simulink model "AUAV_V3_TestSensors_"  (R2015a)
settings: Solver=FixedStepDiscrete  StartTime=0.0  StopTime=10.0  FixedStep=T  RelTol=1e-3
PreLoadFcn:
  | %T = 0.0025;
  | MavlinkBus;
  | mcuInit;
  | % Baro Altitude Computation
  | % =========================
  | basePressure = 98192.64;
  | baseTemp = 288.215;
  | lapseRate = -0.00198122;
  | baseHeight = 0;
values from neighbouring files (symbols this model uses):
  apSampleTime = 0.01    [mcuInit.m]
  latlong_WP = 1    [mcuInit.m]
  mavlink_attitude_t = Simulink.Bus    [MavlinkBusMarcello.m]
  mavlink_gps_raw_int_t = Simulink.Bus    [MavlinkBus.m]    (also in MavlinkBusMarcello.m)
  mavlink_raw_imu_t = Simulink.Bus    [MavlinkBus.m]    (also in MavlinkBusMarcello.m)
  mavlink_scaled_pressure_t = Simulink.Bus    [MavlinkBus.m]    (also in MavlinkBusMarcello.m)
  mavlink_servo_output_raw_t = Simulink.Bus    [MavlinkBusMarcello.m]
  mavlink_sys_status_t = Simulink.Bus    [MavlinkBus.m]    (also in MavlinkBusMarcello.m)
  T = 0.01    [mcuInit.m]
  Xpoints = [0 0]    [mcuInit.m]
  Ypoints = [0 0]    [mcuInit.m]
  Zpoints = [0 0]    [mcuInit.m]
undefined symbols (not defined in the file or in its folder): A0, A14, A15, A2, A3, A4, A5, A6, accBiasRateLimit, B0, bankCommandLimit, barAdjust, baroCutoff, baroCutTemp, cubeAccelGain16405, cubeGyroGain16405, cubeMagGain16405, D0, D11, D7, D8, daLimit, data, daTrimMax, daTrimMin, deLimit, deTrimMax, deTrimMin, drLimit, drTrimMax, drTrimMin, dtLimit, dtTrimMax, dtTrimMin, F2, F3, G0, G13, G15, gaind, GS_location, gyroBiasRateLimit, IC1max, IPStar, ISA_g, Max, maxAcc, MaxDwnPthStar, maxDynPressure, maxEta, mlParamInterface, ms, OC1max, P112, P125, P127, P16, P20, P21, P30 ... (+26)
undefined symbols (not defined in the file): baroOffset, baroScale, barTGain1, barTGain2, barTMean1, barTMean2, bda, bde, bdr, bdt, bICda, bICde, bICdr, bICdt, derivativesConstant, lowRateSensorCutoff, mainSensorCutoff, mda, mde, mdr, mdt, mICda, mICde, mICdr, mICdt, pitotOffset, pitotScale, pitTGain1, pitTGain2, pitTMean1, pitTMean2, powerOffset, powerScale, pressureSensorCutoff, tempOffset, tempScale, vzCutoff, xCutoff, yCutoff
libraries: MCHP_Blockset x150, simulink x84, SLUGS_Library x31, aerolibconvert2 x6, aerolibutil x4, aerolibtransform2 x3, dspmtrx3 x2, aerolibobsolete x2
(part 1 of 20)
Description:
  | Rapid Prototyping model.
  | Require the MPLAB Blockset for Simulink v3.30 or above. [http://www.microchip.com/SimulinkBlocks]
  | Author:Avi Manor Based on Lubin Kerhuels work and code from SLUGS
  | 
  | Test Mavlink on AUAV V3 board from Asrovtech. [http://arsovtech.com/?p=1414]
settings Model: Creator=M91449  LastModifiedBy=User
settings DataIOCC: SignalLoggingSaveFormat=ModelDataLogs
settings OptimizationCC: InlineParams=on  InlineInvariantSignals=on  EnhancedBackFolding=on  OptimizeModelRefInitCode=on  LifeSpan=1
settings DebuggingCC: UnderspecifiedInitializationDetection=Classic  MergeDetectMultiDrivingBlocksExec=none  SolverPrmCheckMsg=warning  MultiTaskDSMMsg=none  FcnCallInpInsideContextMsg=EnableAllAsWarning
settings HardwareCC: ProdBitPerInt=16  ProdBitPerPointer=16  ProdLargestAtomicInteger=Integer  ProdIntDivRoundTo=Zero  ProdEndianess=LittleEndian  ProdWordSize=16  ProdHWDeviceType=Generic->Custom
settings RTWCC: SystemTargetFile=MCHP_dsPIC_stf.tlc  GenCodeOnly=on  TemplateMakefile=MCHP_dsPIC.tmf  Description=Microchip Embedded Target PIC24 dsPIC30 dsPIC33 (real-time)  CustomHeaderCode="#include \"MavlinkComm.h\""
settings RTWCC: CustomSourceCode=|
  | #include "gpsPort.h"
  | #include "MavlinkComm.h"
settings RTWCC: CustomInclude=|
  | mavlink/include/slugs
  | clib\
settings RTWCC: CustomSource=|
  | clib/circBuffer.c
  | clib/gpsPort.c
  | clib/gpsUblox.c
  | clib/MavlinkComm.c
  | clib/apUtils.c
  | clib/mavlinkCommsControlMcu.c
  | clib/mavlinkControlMcu.c
  | clib/mavlinkSensorMcu.c
  | clib/updateControlMcuState.c
  | clib/updateSensorMcuState.c
  | clib/novatel.c
  | clib/navSupport.c
  | clib/hil.c
  | clib/adisCube16405.c
settings RTWCC: CustomInitializer=|
  | uartBufferInit();
  | uartMavlinkBufferInit ();
  | InitParameterInterface();
settings CodeAppCC: IgnoreCustomStorageClasses=off  InternalIdentifier=Classic
settings STFCustomTargetCC: TargetLibSuffix=_lib.a  GenerateSampleERTMain=off  IncludeMdlTerminateFcn=off  CombineOutputUpdateFcns=on  SuppressErrorStatus=on  SupportContinuousTime=off  SupportNonInlinedSFcns=on  SupportVariableSizeSignals=off  SystemTargetFile=MCHP_dsPIC_stf.tlc
settings ERTTargetCC: TargetLibSuffix=_lib.a  GenerateSampleERTMain=off  IncludeMdlTerminateFcn=off  SuppressErrorStatus=on  SupportContinuousTime=off  SupportNonInlinedSFcns=on  SupportVariableSizeSignals=off  ExtModeMexFile=ext_serial_win32_comm_no_acks_rtt  ExtModeMexArgs=1 4 57600  ERTSrcFileBannerTemplate=MCHP_dsPIC_code_template.cgt  ERTHdrFileBannerTemplate=MCHP_dsPIC_code_template.cgt  ERTDataSrcFileTemplate=MCHP_dsPIC_code_template.cgt  ERTDataHdrFileTemplate=MCHP_dsPIC_code_template.cgt  ERTCustomFileTemplate=MCHP_main.tlc

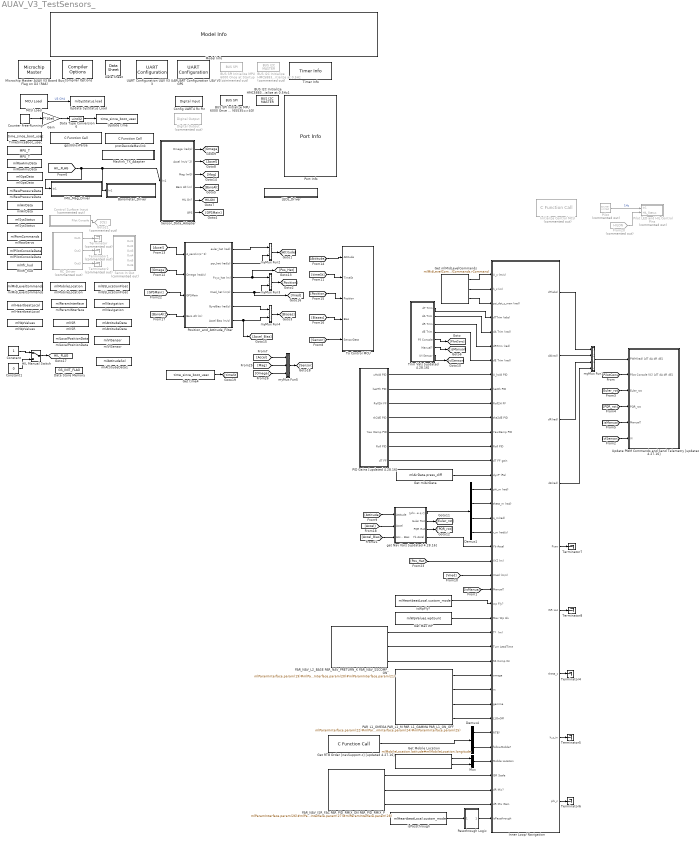
== system AUAV_V3_TestSensors_ ==
  " gpsUbloxParse" : MCHP_Blockset/User Functions/C Function Call  ParseFilesChkbx=on  ListFunctions1=Custom Function  Function1=void gpsUbloxParse(void)  AddHeaderDeclaration=on  Function1Type=when block is updated (default)  FctReturnBlockOut=on  DataCollected="s.chksm=reshape({ '638503-Feb-2015 20:58:10','251913-Sep-2016 12:15:14','1628414-Sep-2016 10:06:29','3596013-Sep-2016 14:21:45','360317-Jun-2016 15:34:16','7112612-Sep-2016 14:50:45','954931-Aug-2016 15:03:40','295329-Aug-2016 11:32:53','268124-Jun-2016 00:23:34','556017-Jun-2016 15:34:16','963217-Jun-2016 15:34:16','1086024-Jun-2016 00:23:34','358817-Jun-2016 15:34:16','985917-Jun-2016 15:34:16','481613-Sep-2016 14:21:38'},1,15);s.File1=reshape({ '  void  newCircBuffer(CBRef cB)','  void  freeCircBuffer(CBRef* cB)','  void  freeCircBuffer(CBRef* cB)',' unsigned int  getLength(CBRef cB)','  int  readHead(CBRef cB)','  int  readTail(CBRef cB)',' unsigned char  peak(CBRef cB)',' unsigned char  readFront(CBRef cB)',' unsigned char  writeBack(CBRef cB, unsigned char data)','  void  makeEmpty(CBRef cB)','  void  printCircBuf(CBRef cB)'},1,11);s.File2=reshape({ '  void  uartBufferInit(void)','  void  __attribute__((__interrupt__, no_auto_psv)) _U4RXInterrupt(void)','  void  getGPSRawData(unsigned char* gpsBuffer)',' unsigned char  isGPSNovatel(void)'},1,4);s.File3=reshape({ '  char  hex2char(char halfhex)','  float  degMinToDeg(unsigned char degrees, float minutes)',' unsigned char  gpsUbloxSeparate(unsigned char* outStream)','  void  gpsUbloxParse(void)','  void  getGpsUbloxMainData(float* data)','  char  gpSmbl(char symbl)',' unsigned char  myTokenizer(char* stringToTokenize, char token, char * returnToken)','  void  parseRMC(unsigned char* stream)','  void  parseGGA(unsigned char* stream)',' unsigned char  getChecksum(unsigned char* sentence, unsigned char size)','  void  gpsDebugMsg(unsigned char buf)'},1,11);s.File4=reshape({ '  void  uartMavlinkBufferInit(void)','  void __attribute__((__interrupt__,__auto_psv__)) _U1RXInterrupt(void)','  uint8_t  isFinite(float s)','  void  InitParameterInterface(void)','  void  protDecodeMavlink(void)','  uint16_t  MissionInterfaceResponse(uint8_t system_id, uint8_t component_id)','  uint16_t  ParameterInterfaceResponse(uint8_t system_id, uint8_t component_id)','  uint16_t  PackHeartBeat(uint8_t system_id, uint8_t component_id)','  uint16_t  PackTextMsg(uint8_t system_id, uint8_t component_id, unsigned char buf)','  uint16_t  PackRawIMU(uint8_t system_id, uint8_t component_id, mavlink_raw_imu_t mlRawIMUData ,uint32_t time_usec)','  uint16_t  PackGpsRawInt(uint8_t system_id, uint8_t component_id, mavlink_gps_raw_int_t mlRawGpsDataInt)','  uint16_t  PackScaledPressure(uint8_t system_id, uint8_t component_id, mavlink_scaled_pressure_t mlAirData ,uint32_t time_usec)','  uint16_t  PackSysStatus(uint8_t system_id, uint8_t component_id, mavlink_sys_status_t mlSysStatus)','  uint16_t  PackRawServo(uint8_t system_id, uint8_t component_id, mavlink_servo_output_raw_t mlPwmCommands ,uint32_t time_usec)','  uint16_t  PackRawRC(uint8_t system_id, uint8_t component_id, mavlink_rc_channels_raw_t mlRC_Commands ,uint32_t time_usec)','  uint16_t  PackVFR_HUD(uint8_t system_id, uint8_t component_id, mavlink_vfr_hud_t mlVfr_hud ,uint32_t time_usec)','  char  sendQGCDebugMessage(const char * dbgMessage, char severity, unsigned char* bytesToAdd, char positionStart)','  void  TxN_Data_OverU1(uint16_t N)'},1,18);s.File5=reshape({ '  float  myAtan2(float num, float denom)','  float  myPow(float x, float toTheN)','  float  mySqrt(float x)','  float  myAbs(float x)','  float  myAtan(float x)','  float  myAsin(float x)','  float  mySin(float x)','  float  myCos(float x)','  float  myTan(float x)','  float  myAcos(float x)','  float  myExp(float x)','  void  hugeDelay(void)','  void  smallDelay(void)','  void  tinyDelay(void)','  void  printToUart2(const char *fmt, ...)'},1,15);s.File6=reshape({ '  void  sendTelemetryMavlink(unsigned char* dataOut)','  void  uart2Init(void)','  void  gsRead(unsigned char* gsChunk)','  void  prepareTelemetryMavlink(unsigned char* dataOut)','  void  prepareTelemetryMavlink(unsigned char* dataOut)','  void  sendTelemetryMavlink(unsigned char* dataOut)','  void  copyBufferToDMA1(unsigned char size)','  void  send2GS(unsigned char* protData)','  uint8_t  clearWaypointsFrom(uint8_t startingWp)','  void  addMessageToSpiOut(mavlink_message_t* msg)'},1,10);s.File7={ '  void  populateParameterInterface(void)'};s.File8={ '  void  mavlinkInit(void)'};s.File9=reshape({ '  void  updatePWM(unsigned short * PWMData)','  void  updatePWMTrim(unsigned short PWMData, unsigned char channel)','  void  updateLoad(uint8_t mcuLoad)','  void  updateEuler(float* newEuler)','  void  updatePQR(float* newPQR)',' unsigned char  getHilOnOff(void)','  uint8_t  getLightsOnOff(void)','  uint8_t  getLightsDayNight(void)','  void  updateVISensor(uint16_t* data)','  void  updatePTZ(int16_t* ptz)'},1,10);s.File10=reshape({ '  void  updateRawADCData(int16_t* adcData)','  void  updateAirData(float* airData)','  void  updateLoadData(uint8_t load, uint16_t mvPower)','  void  updateAttitude(float * attitudeData)','  void  getGSLocation(float* altLatLon)','  void  updateTimeStamp(uint32_t timeSt)','  void  updatePosition(float * posData)','  void  updatePilotConsole(uint16_t * pilData)','  void  updateDiagnosticFl(float* diagFl)','  void  updateDiagnosticSh(int16_t* diagSh)','  void  updateBias(float * biasData)','  void  updateSensorData(float* sens)','  uint8_t  isFixValid(void)','  void  updateSensorDiag(float* diag)'},1,14);s.File11=reshape({ '  void  gpsInit(void)','  void  gpsParse(uint8_t* dataStream)','  void  updateStatus(uint8_t* completeMessage)','  void  updatePositionData(uint8_t* completeMessage)','  void  updateVelocityData(uint8_t* completeMessage)','  void  updateTimeData(uint8_t* completeMessage)','  void  getGpsMainData(float* data)','  uint32_t  CRC32Value(int32_t i)','  uint32_t  CalculateBlockCRC32(uint32_t ulCount, uint8_t *ucBuffer)','  uint16_t  charsToUint16(uint8_t* data)','  uint32_t  charsToUint32(uint8_t* data)','  float  charsToFloat(uint8_t* data)','  double  charsToDouble(uint8_t* data)'},1,13);s.File12=reshape({ '  void  getMidLevelCommands(float* commands)',' unsigned char  isApManual(uint16_t failsafe)','  float  getParamIdx(unsigned char idx)','  void  getRangeOfParams(uint8_t startIdx, uint8_t endIdx, float* parameters)','  float  getDynamic(void)','  void  getAttitude(float* attitude)','  void  getXYZ(float* xyz)','  void  getVned(float* xyz)','  uint8_t  getMaxWp(void)',' unsigned char  isWpFly(void)',' unsigned char  isPassthrough(void)','  void  setDiagnosticFloat(float * flValues)','  void  setDiagnosticShort(int16_t* shValues)','  void  getWP(unsigned char idx, float* WPpos)','  void  setLogFloat1(float * flValues)','  void  setLogFloat2(float * flValues)',' unsigned char  getApControlType(void)',' unsigned char  getPassValues(uint8_t* pasVals)','  void  setCurrentCommands(float airSpeed)','  void  getCurrentGPSPos(float* latLonAlt)','  void  setNavLong(float* values)','  void  setNavLat(float* values)','  void  setNavNav(float* values)','  void  getAccels(float * accels)','  void  getAccBias(float * bias)','  void  getRTB(uint8_t* rtb)','  void  getMobileLocation(float* loc)','  uint8_t  getNavMode(void)','  void  getISRLocation(float* loc)','  uint8_t  getISRCameraOption1(void)',' unsigned short  meanFilter5(unsigned short * values)','  uint8_t  justEnabled(uint8_t enableValue, uint8_t index)',' unsigned char  quickSort(unsigned short *arr, char elements)'},1,33);s.File13=reshape({ '  void  hilRead(unsigned char* hilChunk)','  void  hil_getRawRead(short * rawData)','  void  hil_getVned(float* vned)','  void  hil_getEuler(float* euler)','  void  hil_getRates(float* pqr)','  void  hil_getXYZ(float* xyz)',' unsigned int  hil_getTs(void)','  void  protDecodeHil(uint8_t* dataIn)'},1,8);s.File14=reshape({ '  void  cubeInit(void)','  void  getCubeData(short * cubeData)','  void  updateCubeData(void)','  int16_t  averageData(int16_t* theData, uint8_t count)',' unsigned short  write2Cube(unsigned short data2Send)','  void  __attribute__((interrupt, no_auto_psv)) _T5Interrupt(void)','  short  convert14BitToShort(short wordData)','  short  convert12BitToShort(short wordData)',' unsigned char  isCube16405(void)'},1,9);s.File15=reshape({ '  void  uartMavlinkBufferInit(void)','  uint16_t  PackHeartBeat(uint8_t system_id, uint8_t component_id)','  uint16_t  PackRawRC(uint8_t system_id, uint8_t component_id, mavlink_rc_channels_raw_t mlRC_Commands, uint32_t time_usec)','  uint16_t  PackVFR_HUD(uint8_t system_id, uint8_t component_id, mavlink_vfr_hud_t mlVfr_hud, uint32_t time_usec)','  uint16_t  PackRawIMU(uint8_t system_id, uint8_t component_id, mavlink_raw_imu_t mlRawIMUData ,uint32_t time_usec)','  char  sendQGCDebugMessage(const char * dbgMessage, char severity, unsigned char* bytesToAdd, char positionStart)','  uint16_t  PackGpsRawInt(uint8_t system_id, uint8_t component_id, mavlink_gps_raw_int_t mlRawGpsDataInt)','  uint16_t  PackScaledPressure(uint8_t system_id, uint8_t component_id, mavlink_scaled_pressure_t mlAirData, uint32_t time_usec)','  uint16_t  PackSysStatus(uint8_t system_id, uint8_t component_id, mavlink_sys_status_t mlSysStatus)'},1,9);"  ORDERING=None  SampleTime=0.5  MCHP_MASTERLINK=|  PinDigitalInput=[]  PinDigitalOutput=[]  PinAnalogInput=[]
      | AUAV_V3_TestSensors_/Microchip Master
      | AUAV V3 Board
      | Busy Flag on D2 (RA6)
  " protDecodeMavlink" : MCHP_Blockset/User Functions/C Function Call  ParseFilesChkbx=on  ListFunctions1=Custom Function  Function1=void protDecodeMavlink(void)  AddHeaderDeclaration=off  Function1Type=when block is updated (default)  FctReturnBlockOut=on  DataCollected="s.chksm=reshape({ '638503-Feb-2015 20:58:10','251913-Sep-2016 12:15:14','1628414-Sep-2016 10:06:29','3754120-Sep-2016 14:41:10','360317-Jun-2016 15:34:16','7114620-Sep-2016 10:38:54','954931-Aug-2016 15:03:40','296127-Sep-2016 09:37:43','268124-Jun-2016 00:23:34','556017-Jun-2016 15:34:16','963217-Jun-2016 15:34:16','1086024-Jun-2016 00:23:34','372414-Sep-2016 14:01:55','998814-Sep-2016 11:55:45','509015-Sep-2016 09:12:19'},1,15);s.File1=reshape({ '  void  newCircBuffer(CBRef cB)','  void  freeCircBuffer(CBRef* cB)','  void  freeCircBuffer(CBRef* cB)',' unsigned int  getLength(CBRef cB)','  int  readHead(CBRef cB)','  int  readTail(CBRef cB)',' unsigned char  peak(CBRef cB)',' unsigned char  readFront(CBRef cB)',' unsigned char  writeBack(CBRef cB, unsigned char data)','  void  makeEmpty(CBRef cB)','  void  printCircBuf(CBRef cB)'},1,11);s.File2=reshape({ '  void  uartBufferInit(void)','  void  __attribute__((__interrupt__, no_auto_psv)) _U4RXInterrupt(void)','  void  getGPSRawData(unsigned char* gpsBuffer)',' unsigned char  isGPSNovatel(void)'},1,4);s.File3=reshape({ '  char  hex2char(char halfhex)','  float  degMinToDeg(unsigned char degrees, float minutes)',' unsigned char  gpsUbloxSeparate(unsigned char* outStream)','  void  gpsUbloxParse(void)','  void  getGpsUbloxMainData(float* data)','  char  gpSmbl(char symbl)',' unsigned char  myTokenizer(char* stringToTokenize, char token, char * returnToken)','  void  parseRMC(unsigned char* stream)','  void  parseGGA(unsigned char* stream)',' unsigned char  getChecksum(unsigned char* sentence, unsigned char size)','  void  gpsDebugMsg(unsigned char buf)'},1,11);s.File4=reshape({ '  void  uartMavlinkBufferInit(void)','  void __attribute__((__interrupt__,__auto_psv__)) _U1RXInterrupt(void)','  uint8_t  isFinite(float s)','  void  InitParameterInterface(void)','  void  protDecodeMavlink(void)','  uint16_t  MissionInterfaceResponse(uint8_t system_id, uint8_t component_id)','  uint16_t  ParameterInterfaceResponse(uint8_t system_id, uint8_t component_id)','  uint16_t  PackHeartBeat(uint8_t system_id, uint8_t component_id)','  uint16_t  PackTextMsg(uint8_t system_id, uint8_t component_id, unsigned char buf)','  uint16_t  PackRawIMU(uint8_t system_id, uint8_t component_id, mavlink_raw_imu_t mlRawIMUData ,uint32_t time_usec)','  uint16_t  PackGpsRawInt(uint8_t system_id, uint8_t component_id, mavlink_gps_raw_int_t mlRawGpsDataInt ,uint32_t time_usec)','  uint16_t  PackScaledPressure(uint8_t system_id, uint8_t component_id, mavlink_scaled_pressure_t mlAirData ,uint32_t time_usec)','  uint16_t  PackSysStatus(uint8_t system_id, uint8_t component_id, mavlink_sys_status_t mlSysStatus)','  uint16_t  PackRawServo(uint8_t system_id, uint8_t component_id, mavlink_servo_output_raw_t mlPwmCommands ,uint32_t time_usec)','  uint16_t  HIL_PackRawServo(uint8_t system_id, uint8_t component_id, mavlink_servo_output_raw_t mlPwmCommands ,uint32_t time_usec)','  uint16_t  PackRawRC(uint8_t system_id, uint8_t component_id, mavlink_rc_channels_raw_t mlRC_Commands ,uint32_t time_usec)','  uint16_t  PackVFR_HUD(uint8_t system_id, uint8_t component_id, mavlink_vfr_hud_t mlVfr_hud ,uint32_t time_usec)','  char  sendQGCDebugMessage(const char * dbgMessage, char severity, unsigned char* bytesToAdd, char positionStart)','  void  TxN_Data_OverU1(uint16_t N)','  void  TxN_Data_OverU4(uint16_t N)'},1,20);s.File5=reshape({ '  float  myAtan2(float num, float denom)','  float  myPow(float x, float toTheN)','  float  mySqrt(float x)','  float  myAbs(float x)','  float  myAtan(float x)','  float  myAsin(float x)','  float  mySin(float x)','  float  myCos(float x)','  float  myTan(float x)','  float  myAcos(float x)','  float  myExp(float x)','  void  hugeDelay(void)','  void  smallDelay(void)','  void  tinyDelay(void)','  void  printToUart2(const char *fmt, ...)'},1,15);s.File6=reshape({ '  void  sendTelemetryMavlink(unsigned char* dataOut)','  void  uart2Init(void)','  void  gsRead(unsigned char* gsChunk)','  void  prepareTelemetryMavlink(unsigned char* dataOut)','  void  prepareTelemetryMavlink(unsigned char* dataOut)','  void  sendTelemetryMavlink(unsigned char* dataOut)','  void  copyBufferToDMA1(unsigned char size)','  void  send2GS(unsigned char* protData)','  uint8_t  clearWaypointsFrom(uint8_t startingWp)','  void  addMessageToSpiOut(mavlink_message_t* msg)'},1,10);s.File7={ '  void  populateParameterInterface(void)'};s.File8={ '  void  mavlinkInit(void)'};s.File9=reshape({ '  void  updatePWM(unsigned short * PWMData)','  void  updatePWMTrim(unsigned short PWMData, unsigned char channel)','  void  updateLoad(uint8_t mcuLoad)','  void  updateEuler(float* newEuler)','  void  updatePQR(float* newPQR)',' unsigned char  getHilOnOff(void)','  uint8_t  getLightsOnOff(void)','  uint8_t  getLightsDayNight(void)','  void  updateVISensor(uint16_t* data)','  void  updatePTZ(int16_t* ptz)'},1,10);s.File10=reshape({ '  void  updateRawADCData(int16_t* adcData)','  void  updateAirData(float* airData)','  void  updateLoadData(uint8_t load, uint16_t mvPower)','  void  updateAttitude(float * attitudeData)','  void  getGSLocation(float* altLatLon)','  void  updateTimeStamp(uint32_t timeSt)','  void  updatePosition(float * posData)','  void  updatePilotConsole(uint16_t * pilData)','  void  updateDiagnosticFl(float* diagFl)','  void  updateDiagnosticSh(int16_t* diagSh)','  void  updateBias(float * biasData)','  void  updateSensorData(float* sens)','  uint8_t  isFixValid(void)','  void  updateSensorDiag(float* diag)'},1,14);s.File11=reshape({ '  void  gpsInit(void)','  void  gpsParse(uint8_t* dataStream)','  void  updateStatus(uint8_t* completeMessage)','  void  updatePositionData(uint8_t* completeMessage)','  void  updateVelocityData(uint8_t* completeMessage)','  void  updateTimeData(uint8_t* completeMessage)','  void  getGpsMainData(float* data)','  uint32_t  CRC32Value(int32_t i)','  uint32_t  CalculateBlockCRC32(uint32_t ulCount, uint8_t *ucBuffer)','  uint16_t  charsToUint16(uint8_t* data)','  uint32_t  charsToUint32(uint8_t* data)','  float  charsToFloat(uint8_t* data)','  double  charsToDouble(uint8_t* data)'},1,13);s.File12=reshape({ '  void  getMidLevelCommands(float* commands)',' unsigned char  isApManual(uint16_t failsafe)','  float  getParamIdx(unsigned char idx)','  void  getRangeOfParams(uint8_t startIdx, uint8_t endIdx, float* parameters)','  float  getDynamic(void)','  void  getAttitude(float* attitude)','  void  getXYZ(float* xyz)','  void  getVned(float* xyz)','  uint8_t  getMaxWp(void)',' unsigned char  isWpFly(void)',' unsigned char  isPassthrough(void)','  void  setDiagnosticFloat(float * flValues)','  void  setDiagnosticShort(int16_t* shValues)','  void  getWP(unsigned char idx, float* WPpos)','  void  setLogFloat1(float * flValues)','  void  setLogFloat2(float * flValues)',' unsigned char  getApControlType(void)',' unsigned char  getPassValues(uint8_t* pasVals)','  void  setCurrentCommands(float airSpeed)','  void  getCurrentGPSPos(float* latLonAlt)','  void  setNavLong(float* values)','  void  setNavLat(float* values)','  void  setNavNav(float* values)','  void  getAccels(float * accels)','  void  getAccBias(float * bias)','  void  getRTB(uint8_t* rtb)','  void  getMobileLocation(float* loc)','  uint8_t  getNavMode(void)','  void  getISRLocation(float* loc)','  uint8_t  getISRCameraOption1(void)',' unsigned short  meanFilter5(unsigned short * values)','  uint8_t  justEnabled(uint8_t enableValue, uint8_t index)',' unsigned char  quickSort(unsigned short *arr, char elements)'},1,33);s.File13=reshape({ '  void  hilRead(unsigned char* hilChunk)','  void  hil_getRawRead(short * rawData)','  void  hil_getVned(float* vned)','  void  hil_getEuler(float* euler)','  void  hil_getRates(float* pqr)','  void  hil_getXYZ(float* xyz)',' unsigned int  hil_getTs(void)','  void  protDecodeHil(uint8_t* dataIn)'},1,8);s.File14=reshape({ '  void  cubeInit(void)','  void  getCubeData(short * cubeData)','  void  updateCubeData(void)','  int16_t  averageData(int16_t* theData, uint8_t count)',' unsigned short  write2Cube(unsigned short data2Send)','  short  convert14BitToShort(short wordData)','  short  convert12BitToShort(short wordData)',' unsigned char  isCube16405(void)'},1,8);s.File15=reshape({ '  void  uartMavlinkBufferInit(void)','  uint16_t  PackHeartBeat(uint8_t system_id, uint8_t component_id)','  uint16_t  PackRawServo(uint8_t system_id, uint8_t component_id, mavlink_servo_output_raw_t mlPwmCommands ,uint32_t time_usec)','  uint16_t  HIL_PackRawServo(uint8_t system_id, uint8_t component_id, mavlink_servo_output_raw_t mlPwmCommands ,uint32_t time_usec)','  uint16_t  PackRawRC(uint8_t system_id, uint8_t component_id, mavlink_rc_channels_raw_t mlRC_Commands, uint32_t time_usec)','  uint16_t  PackVFR_HUD(uint8_t system_id, uint8_t component_id, mavlink_vfr_hud_t mlVfr_hud, uint32_t time_usec)','  uint16_t  PackRawIMU(uint8_t system_id, uint8_t component_id, mavlink_raw_imu_t mlRawIMUData ,uint32_t time_usec)','  char  sendQGCDebugMessage(const char * dbgMessage, char severity, unsigned char* bytesToAdd, char positionStart)','  uint16_t  PackGpsRawInt(uint8_t system_id, uint8_t component_id, mavlink_gps_raw_int_t mlRawGpsDataInt, uint32_t time_usec)','  uint16_t  PackScaledPressure(uint8_t system_id, uint8_t component_id, mavlink_scaled_pressure_t mlAirData, uint32_t time_usec)','  uint16_t  PackSysStatus(uint8_t system_id, uint8_t component_id, mavlink_sys_status_t mlSysStatus)'},1,11);"  ORDERING=None  SampleTime=0.2  MCHP_MASTERLINK=|  PinDigitalInput=[]  PinDigitalOutput=[]  PinAnalogInput=[]
      | AUAV_V3_TestSensors_/Microchip Master
      | AUAV V3 Board
      | Busy Flag on D2 (RA6)
  BUS I2C Initialize HMC5883 re-initialize at 0.5Hz : MCHP_Blockset/BUS I2C/BUS I2C MASTER  Commented=on  I2CRef=2  I2C_IntPriority=6  I2Csequence_txt="Initial-Configuration$     ---     $Start$Write Address:{[0x1E]}    % HMC5883L Address$Write Data (x1)  Write:{[0x00 0x78 0x00 0x00]}      % Configure$Stop"  I2Csequence_num=[BFF0000000000000 40E0600000000000 41186A0000000000 4118666E3C87173F]$[4070000000000000]$[3FF0000000000000 40E0200000000000 40F86A0000000000 40F866E066594CA2]$[4040000000000000 0000000000000000 0000000000000000 403E000000000000]$[4050000000000000 3FF0000000000000 0000000000000000 0000000000000000 405E000000000000 0000000000000000 0000000000000000]$[4000000000000000 40E0600000000000 40F86A0000000000 40F866E066594CA2]  InitialConfigurationNum=0  PIN_SDA_TXT=A3 / Pin[59]  PIN_SCL_TXT=A2 / Pin[58]  S_INPUT="[5  5]"  S_OUTPUT=[5]  S_INPUT_Size="[2  2]"  S_OUTPUT_Size=[4]  BlockingMode=off  SampleTime=.5  MCHP_MASTERLINK=|  MCHP_PORT={I2C 2 Clock}{SCL2}13:0:A2;{I2C 2 SDA}{SDA2}13:0:A3;  ORDERING=0
      | AUAV_V3_TestSensors/Microchip Master
      | AUAV V3 Board
      | Busy Flag on D2 (RA6)
  BUS I2C Initialize HMC5883 re-initialize at 0.5Hz1 : MCHP_Blockset/BUS I2C/BUS I2C MASTER  I2CRef=2  I2C_IntPriority=6  I2Csequence_txt="Initial-Configuration$     ---     $Start$Write Address:{[0x1E]}    % HMC5883L Address$Write Data (x1)  Write:{[0x00 0x78 0x00 0x00]}      % Configure$Stop"  I2Csequence_num=[BFF0000000000000 40E0600000000000 40F86A0000000000 410065D9C7810E65]$[4070000000000000]$[3FF0000000000000 40E0200000000000 40F86A0000000000 40F866E066594CA2]$[4040000000000000 0000000000000000 0000000000000000 403E000000000000]$[4050000000000000 3FF0000000000000 0000000000000000 0000000000000000 405E000000000000 0000000000000000 0000000000000000]$[4000000000000000 40E0600000000000 40F86A0000000000 40F866E066594CA2]  InitialConfigurationNum=0  PIN_SDA_TXT=A3 / Pin[59]  PIN_SCL_TXT=A2 / Pin[58]  S_INPUT="[5  5]"  S_OUTPUT=[5]  S_INPUT_Size="[2  2]"  S_OUTPUT_Size=[4]  BlockingMode=off  SampleTime=.5  MCHP_MASTERLINK=|  MCHP_PORT={I2C 2 Clock}{SCL2}13:0:A2;{I2C 2 SDA}{SDA2}13:0:A3;  ORDERING=0
      | AUAV_V3_TestSensors/Microchip Master
      | AUAV V3 Board
      | Busy Flag on D2 (RA6)
  BUS SPI Initialize MPU 6000 Once at Startup : MCHP_Blockset/BUS SPI/BUS SPI  Commented=on  SPIRef=1  DMA="[0  2  3]"  SPI_IntPriority=5  SPIsequence_txt="Initial-Configuration$     ---     $Set Port E4 / Pin[100] to 1    % /CS$Delay of 0.01(s)$Set Port E4 / Pin[100] to 0    % /CS$Write only (x1)  Write:{[0x6B80]}      % PWR_MGMT_1, BIT_H_RESET$Set Port E4 / Pin[100] to 1    % /CS$Delay of 0.06(s)$Set Port E4 / Pin[100] to 0    % /CS$Write only (x1)  Write:{[0x6B01]}      % PWR_MGMT_1, MPU_CLK_SEL_PLLGYROZ - PLL with X axis gyroscope reference$Set Port E4 / Pin[100] to 1    % /CS$Delay of 0.01(s)$Set Port E4 / Pin[100] to 0    % /CS$Write only (x1)  Write:{[0x6A10]}      % conf Pow Mngt 1$Set Port E4 / Pin[100] to 1    % /CS$Delay of 0.01(s)$Set Port E4 / Pin[100] to 0    % /CS$Write only (x1)  Write:{[0x1904]}      % Sample rate = 200Hz  Fsample= 1Khz/(N+1) = 200Hz$Set Port E4 / Pin[100] to 1    % /CS$Delay of 0.01(s)$Set Port E4 / Pin[100] to 0    % /CS$Write only (x1)  Write:{[0x1A03]}      % LPF - Gyro 42Hz 4.8mS delay - Accel 44Hz 4.9mS delay$Set Port E4 / Pin[100] to 1    % /CS$Delay of 0.01(s)$Set Port E4 / Pin[100] to 0$Write only (x1)  Write:{[0x1B08]}      % Gyro scale 500º/s$Set Port E4 / Pin[100] to 1"  SPIsequence_num=[BFF0000000000000 4091D00000000000 0000000000000000 40E0000000000000 4116409C00000000 4116409D55555555]$[4070000000000000]$[4010000000000000 4051000000000000 3FF0000000000000]$[4020000000000000 3F847AE147AE147B]$[4010000000000000 4051000000000000 0000000000000000]$[3FF0000000000000 3FF0000000000000 0000000000000000 40DAE00000000000]$[4010000000000000 4051000000000000 3FF0000000000000]$[4020000000000000 3FAEB851EB851EB8]$[4010000000000000 4051000000000000 0000000000000000]$[3FF0000000000000 3FF0000000000000 0000000000000000 40DAC04000000000]$[4010000000000000 4051000000000000 3FF0000000000000]$[4020000000000000 3F847AE147AE147B]$[4010000000000000 4051000000000000 0000000000000000]$[3FF0000000000000 3FF0000000000000 0000000000000000 40DA840000000000]$[4010000000000000 4051000000000000 3FF0000000000000]$[4020000000000000 3F847AE147AE147B]$[4010000000000000 4051000000000000 0000000000000000]$[3FF0000000000000 3FF0000000000000 0000000000000000 40B9040000000000]$[4010000000000000 4051000000000000 3FF0000000000000]$[4020000000000000 3F847AE147AE147B]$[4010000000000000 4051000000000000 0000000000000000]$[3FF0000000000000 3FF0000000000000 0000000000000000 40BA030000000000]$[4010000000000000 4051000000000000 3FF0000000000000]$[4020000000000000 3F847AE147AE147B]$[4010000000000000 4051000000000000 0000000000000000]$[3FF0000000000000 3FF0000000000000 0000000000000000 40BB080000000000]$[4010000000000000 4051000000000000 3FF0000000000000]  PIN_SDI_TXT=E3 / P83 / Pin[99]  PIN_SDO_TXT=E2 / P82 / Pin[98]  PIN_SCK_TXT=G15 / P127 / Pin[1]  PIN_SS_TXT=B0 / Pin[21]  S_INPUT="[5  5]"  S_OUTPUT=[5]  S_INPUT_Size="[2  2]"  S_OUTPUT_Size=[4]  BlockingMode=off  SampleTime=inf  MCHP_MASTERLINK=|  MCHP_PORT={SPI 1 input}{SDI1}12:0:P83;{SPI 1 output}{SDO1}12:1:P82;{SPI 1 Clock output}{SCK1}12:1:P127;{SPI 1 Digital output}{SPI1-DOU}12:1:E4;{SPI 1 Digital output}{SPI1-DOU}12:1:E4;{SPI 1 Digital output}{SPI1-DOU}12:1:E4;{SPI 1 Digital output}{SPI1-DOU}12:1:E4;{SPI 1 Digital output}{SPI1-DOU}12:1:E4;{SPI 1 Digital output}{SPI1-DOU}12:1:E4;{SPI 1 Digital output}{SPI1-DOU}12:1:E4;{SPI 1 Digital output}{SPI1-DOU}12:1:E4;{SPI 1 Digital output}{SPI1-DOU}12:1:E4;{SPI 1 Digital output}{SPI1-DOU}12:1:E4;{SPI 1 Digital output}{SPI1-DOU}12:1:E4;{SPI 1 Digital output}{SPI1-DOU}12:1:E4;{SPI 1 Digital output}{SPI1-DOU}12:1:E4;  ORDERING=0
      | AUAV_V3_TestSensors/Microchip Master
      | AUAV V3 Board
      | Busy Flag on D2 (RA6)
  BUS SPI Initialize MPU 6000 Once at Startup Gyro:+-500°/s (65535=>1000) Accelero: +-2G (65535=>4G) : MCHP_Blockset/BUS SPI/BUS SPI  SPIRef=1  DMA="[0  2  3]"  SPI_IntPriority=5  SPIsequence_txt="Initial-Configuration$     ---     $Set Port E4 / Pin[100] to 1    % /CS$Delay of 0.01(s)$Set Port E4 / Pin[100] to 0    % /CS$Write only (x1)  Write:{[0x6A80]}      % conf Pow Mngt 1$Set Port E4 / Pin[100] to 1    % /CS$Delay of 0.06(s)$Set Port E4 / Pin[100] to 0    % /CS$Write only (x1)  Write:{[0x6B01]}      % conf Pow Mngt 1$Set Port E4 / Pin[100] to 1    % /CS$Delay of 0.01(s)$Set Port E4 / Pin[100] to 0    % /CS$Write only (x1)  Write:{[0x1B08]}      % Set rate gyro Scaling 500deg$Set Port E4 / Pin[100] to 1    % /CS$Delay of 0.01(s)$Set Port E4 / Pin[100] to 0    % /CS$Write only (x1)  Write:{[0x6A10]}      % conf Pow Mngt 1$Set Port E4 / Pin[100] to 1    % /CS"  SPIsequence_num=[BFF0000000000000 4091D00000000000 0000000000000000 40E0000000000000 4116409C00000000 4116409D55555555]$[4070000000000000]$[4010000000000000 4051000000000000 3FF0000000000000]$[4020000000000000 3F847AE147AE147B]$[4010000000000000 4051000000000000 0000000000000000]$[3FF0000000000000 3FF0000000000000 0000000000000000 40DAA00000000000]$[4010000000000000 4051000000000000 3FF0000000000000]$[4020000000000000 3FAEB851EB851EB8]$[4010000000000000 4051000000000000 0000000000000000]$[3FF0000000000000 3FF0000000000000 0000000000000000 40DAC04000000000]$[4010000000000000 4051000000000000 3FF0000000000000]$[4020000000000000 3F847AE147AE147B]$[4010000000000000 4051000000000000 0000000000000000]$[3FF0000000000000 3FF0000000000000 0000000000000000 40BB080000000000]$[4010000000000000 4051000000000000 3FF0000000000000]$[4020000000000000 3F847AE147AE147B]$[4010000000000000 4051000000000000 0000000000000000]$[3FF0000000000000 3FF0000000000000 0000000000000000 40DA840000000000]$[4010000000000000 4051000000000000 3FF0000000000000]  PIN_SDI_TXT=E3 / P83 / Pin[99]  PIN_SDO_TXT=E2 / P82 / Pin[98]  PIN_SCK_TXT=G15 / P127 / Pin[1]  PIN_SS_TXT=B0 / Pin[21]  S_INPUT="[5  5]"  S_OUTPUT=[5]  S_INPUT_Size="[2  2]"  S_OUTPUT_Size=[4]  BlockingMode=off  SampleTime=inf  MCHP_MASTERLINK=|  MCHP_PORT={SPI 1 input}{SDI1}12:0:P83;{SPI 1 output}{SDO1}12:1:P82;{SPI 1 Clock output}{SCK1}12:1:P127;{SPI 1 Digital output}{SPI1-DOU}12:1:E4;{SPI 1 Digital output}{SPI1-DOU}12:1:E4;{SPI 1 Digital output}{SPI1-DOU}12:1:E4;{SPI 1 Digital output}{SPI1-DOU}12:1:E4;{SPI 1 Digital output}{SPI1-DOU}12:1:E4;{SPI 1 Digital output}{SPI1-DOU}12:1:E4;{SPI 1 Digital output}{SPI1-DOU}12:1:E4;{SPI 1 Digital output}{SPI1-DOU}12:1:E4;{SPI 1 Digital output}{SPI1-DOU}12:1:E4;  ORDERING=0
      | AUAV_V3_TestSensors/Microchip Master
      | AUAV V3 Board
      | Busy Flag on D2 (RA6)
  Barometer_Driver : Subsystem  TreatAsAtomicUnit=on
      settings: RTWFileNameOpts=Use subsystem name
  Compiler Options : MCHP_Blockset/System Configuration/Compiler Options  Priority=1  LATEST_CMPLR=on  COMP_LIST=Dynamic Options  COMP_LIST_TXT=xc16 - v1.26  USE_64BIT_DOUBLE=off  MCHP_MULTITHREAD_COMPILATION=on  MCHP_MASTERLINK=|  OPTIMIZATION_LEVEL=1  MPLAB_LINKLIB=default  MPLAB_LINKLIB1=default  UNROLL_LOOPS=off  OMIT_FRAME_POINTER=off  PROCEDURAL_ABSTRACTION=off  MCONST=in code memory  MDATA=Can use all available memory  MSCALAR=Can use all available memory  MCODE=is more than 32768  HEAP_SIZE=0  OMF=elf  DEBUG_INFO=off  AssemblyListing=off  ProduceHexOutput=on
      | AUAV_V3_TestSensors/Microchip Master
      | AUAV V3 Board
      | Busy Flag on D2 (RA6)
  Config UART4 Rx Pin : MCHP_Blockset/Digital IO/Digital Input  PORT=Dynamic Options  PORT_TXT="E   [ 0 : 9 ]"  PIN=[6]  PACK=off  SIMULTANEOUS=off  ORDERING=None  SampleTime=-1  MCHP_PORT={Digital In}{DIN}2:0:E6;  MCHP_MASTERLINK=|
      | AUAV_V3_TestSensors/Microchip Master
      | AUAV V3 Board
      | Busy Flag on D2 (RA6)
  Constant : Constant
  Constant1 : Constant  Value=0
  Control Surface Input : Subsystem  Commented=on
  Counter Free-Running : simulink/Sources/Counter Free-Running  NumBits=32  tsamp=T
  Data Sheet : MCHP_Blockset/System Info/Data Sheet  DOC_MCHP_Id=33EP512MU810  DOC_FilePath=C:\Users\M91449\AppData\Local\Temp\70616g.pdf  DOC_FileLastCheckTime="[2013             11             10             22              4         17.021]"  cpy_MCHP_Id=33EP512MU810  MCHP_MASTERLINK=|
      | AUAV_V3_TestSensors/Microchip Master
      | AUAV V3 Board
      | Busy Flag on D2 (RA6)
      settings: AttributesFormatString=%<cpy_MCHP_Id>
  Data Store Memory : DataStoreMemory  DataStoreName=GS_INIT_FLAG  ReadBeforeWriteMsg=warning  WriteAfterWriteMsg=warning  WriteAfterReadMsg=warning  InitialValue=1
  Data Type Conversion6 : DataTypeConversion  OutDataTypeStr=uint32
  Demux1 : Demux
  Demux4 : Demux  Outputs=2
  Digital Output : MCHP_Blockset/Digital IO/Digital Output  Commented=on  PORT=Dynamic Options  PORT_TXT="E   [ 0 : 9 ]"  PIN=[5]  PACK=off  SIMULTANEOUS=off  READPREVIOUS=off  ORDERING=None  SampleTime=-1  MCHP_MASTERLINK=|
      | AUAV_V3_TestSensors/Microchip Master
      | AUAV V3 Board
      | Busy Flag on D2 (RA6)
  From20 : From  Commented=on  GotoTag=HILON  TagVisibility=global
  Gain : Gain  Gain=T*10e6
  Get Max WP : DataStoreRead  DialogController=Simulink.DDGSource  DataStoreName=mlWpValues  DataStoreElements=mlWpValues.wpCount
  Get Mobile Location : DataStoreRead  DialogController=Simulink.DDGSource  DataStoreName=mlMobileLocation  DataStoreElements=mlMobileLocation.latitude#mlMobileLocation.longitude
  Get RTB Order [navSupport.c] [updated 4.27.16] : MCHP_Blockset/User Functions/C Function Call  ParseFilesChkbx=off  ListFunctions1=Custom Function  Function1=extern void getRTB(uint8_T* y1);  AddHeaderDeclaration=on  Function1Type=when block is updated (default)  FctReturnBlockOut=on  Fct1BlockOut=y1[2]  DataCollected=0  ORDERING=None  SampleTime=0.01  MCHP_MASTERLINK=|  PinDigitalInput=[]  PinDigitalOutput=[]  PinAnalogInput=[]
      | AUAV_V3_TestSensors_/Microchip Master
      | AUAV V3 Board
      | Busy Flag on D2 (RA6)
  Get mlAirData : DataStoreRead  DialogController=Simulink.DDGSource  DataStoreName=mlAirData  DataStoreElements=mlAirData.press_diff
  Get mlMidLevelCommands : DataStoreRead  DialogController=Simulink.DDGSource  DataStoreName=mlMidLevelCommands  DataStoreElements=mlMidLevelCommands.uCommand#mlMidLevelCommands.hCommand#mlMidLevelCommands.rCommand
  Get time4 : DataStoreRead  DataStoreName=time_since_boot_usec  DataStoreElements=time_since_boot_usec
  Goto21 : Goto  Commented=on  GotoTag=CS
  HIL Manual Switch : ManualSwitch
  IMU_Mag_Driver : Subsystem  TreatAsAtomicUnit=on
      settings: RTWFileNameOpts=Use subsystem name
  Initialize Control MCU : MCHP_Blockset/User Functions/C Function Call  Commented=on  ParseFilesChkbx=on  ListFunctions1=Custom Function  Function1=void controlMCUInit();  AddHeaderDeclaration=on  Function1Type=only once at power-up time  FctReturnBlockOut=on  DataCollected="s.chksm=reshape({ '638503-Feb-2015 20:58:10','219617-Jun-2016 15:34:16','1598516-Aug-2016 15:57:55','3587131-Aug-2016 11:49:56','360317-Jun-2016 15:34:16','7105631-Aug-2016 15:29:43','954931-Aug-2016 15:03:40','295329-Aug-2016 11:32:53','268124-Jun-2016 00:23:34','556017-Jun-2016 15:34:16','963217-Jun-2016 15:34:16','1086024-Jun-2016 00:23:34','358817-Jun-2016 15:34:16','985917-Jun-2016 15:34:16','493729-Aug-2016 10:55:43'},1,15);s.File1=reshape({ '  void  newCircBuffer(CBRef cB)','  void  freeCircBuffer(CBRef* cB)','  void  freeCircBuffer(CBRef* cB)',' unsigned int  getLength(CBRef cB)','  int  readHead(CBRef cB)','  int  readTail(CBRef cB)',' unsigned char  peak(CBRef cB)',' unsigned char  readFront(CBRef cB)',' unsigned char  writeBack(CBRef cB, unsigned char data)','  void  makeEmpty(CBRef cB)','  void  printCircBuf(CBRef cB)'},1,11);s.File2=reshape({ '  void  uartBufferInit(void)','  void  __attribute__((__interrupt__, no_auto_psv)) _U4RXInterrupt(void)','  void  getGPSRawData(unsigned char* gpsBuffer)',' unsigned char  isGPSNovatel(void)'},1,4);s.File3=reshape({ '  char  hex2char(char halfhex)','  float  degMinToDeg(unsigned char degrees, float minutes)',' unsigned char  gpsUbloxSeparate(unsigned char* outStream)','  void  gpsUbloxParse(void)','  void  getGpsUbloxMainData(float* data)','  char  gpSmbl(char symbl)',' unsigned char  myTokenizer(char* stringToTokenize, char token, char * returnToken)','  void  parseRMC(unsigned char* stream)','  void  parseGGA(unsigned char* stream)',' unsigned char  getChecksum(unsigned char* sentence, unsigned char size)'},1,10);s.File4=reshape({ '  void  uartMavlinkBufferInit(void)','  void __attribute__((__interrupt__,__auto_psv__)) _U1RXInterrupt(void)','  uint8_t  isFinite(float s)','  void  InitParameterInterface(void)','  void  protDecodeMavlink(void)','  uint16_t  MissionInterfaceResponse(uint8_t system_id, uint8_t component_id)','  uint16_t  ParameterInterfaceResponse(uint8_t system_id, uint8_t component_id)','  uint16_t  PackHeartBeat(uint8_t system_id, uint8_t component_id)','  uint16_t  PackTextMsg(uint8_t system_id, uint8_t component_id)','  uint16_t  PackRawIMU(uint8_t system_id, uint8_t component_id, mavlink_raw_imu_t mlRawIMUData ,uint32_t time_usec)','  uint16_t  PackGpsRawInt(uint8_t system_id, uint8_t component_id, mavlink_gps_raw_int_t mlRawGpsDataInt ,uint32_t time_usec)','  uint16_t  PackScaledPressure(uint8_t system_id, uint8_t component_id, mavlink_scaled_pressure_t mlAirData ,uint32_t time_usec)','  uint16_t  PackSysStatus(uint8_t system_id, uint8_t component_id, mavlink_sys_status_t mlSysStatus)','  uint16_t  PackRawServo(uint8_t system_id, uint8_t component_id, mavlink_servo_output_raw_t mlPwmCommands ,uint32_t time_usec)','  uint16_t  PackRawRC(uint8_t system_id, uint8_t component_id, mavlink_rc_channels_raw_t mlRC_Commands ,uint32_t time_usec)','  uint16_t  PackVFR_HUD(uint8_t system_id, uint8_t component_id, mavlink_vfr_hud_t mlVfr_hud ,uint32_t time_usec)','  char  sendQGCDebugMessage(const char * dbgMessage, char severity, unsigned char* bytesToAdd, char positionStart)','  void  TxN_Data_OverU1(uint16_t N)'},1,18);s.File5=reshape({ '  float  myAtan2(float num, float denom)','  float  myPow(float x, float toTheN)','  float  mySqrt(float x)','  float  myAbs(float x)','  float  myAtan(float x)','  float  myAsin(float x)','  float  mySin(float x)','  float  myCos(float x)','  float  myTan(float x)','  float  myAcos(float x)','  float  myExp(float x)','  void  hugeDelay(void)','  void  smallDelay(void)','  void  tinyDelay(void)','  void  printToUart2(const char *fmt, ...)'},1,15);s.File6=reshape({ '  void  sendTelemetryMavlink(unsigned char* dataOut)','  void  uart2Init(void)','  void  gsRead(unsigned char* gsChunk)','  void  prepareTelemetryMavlink(unsigned char* dataOut)','  void  prepareTelemetryMavlink(unsigned char* dataOut)','  void  sendTelemetryMavlink(unsigned char* dataOut)','  void  copyBufferToDMA1(unsigned char size)','  void  send2GS(unsigned char* protData)','  void  __attribute__((interrupt, no_auto_psv)) _DMA1Interrupt(void)','  void  __attribute__((__interrupt__, no_auto_psv)) _U2RXInterrupt(void)','  void  __attribute__((interrupt, no_auto_psv)) _U2ErrInterrupt(void)','  uint8_t  clearWaypointsFrom(uint8_t startingWp)','  void  addMessageToSpiOut(mavlink_message_t* msg)'},1,13);s.File7={ '  void  populateParameterInterface(void)'};s.File8={ '  void  mavlinkInit(void)'};s.File9=reshape({ '  void  updatePWM(unsigned short * PWMData)','  void  updatePWMTrim(unsigned short PWMData, unsigned char channel)','  void  updateLoad(uint8_t mcuLoad)','  void  updateEuler(float* newEuler)','  void  updatePQR(float* newPQR)',' unsigned char  getHilOnOff(void)','  uint8_t  getLightsOnOff(void)','  uint8_t  getLightsDayNight(void)','  void  updateVISensor(uint16_t* data)','  void  updatePTZ(int16_t* ptz)'},1,10);s.File10=reshape({ '  void  updateRawADCData(int16_t* adcData)','  void  updateAirData(float* airData)','  void  updateLoadData(uint8_t load, uint16_t mvPower)','  void  updateAttitude(float * attitudeData)','  void  getGSLocation(float* altLatLon)','  void  updateTimeStamp(uint32_t timeSt)','  void  updatePosition(float * posData)','  void  updatePilotConsole(uint16_t * pilData)','  void  updateDiagnosticFl(float* diagFl)','  void  updateDiagnosticSh(int16_t* diagSh)','  void  updateBias(float * biasData)','  void  updateSensorData(float* sens)','  uint8_t  isFixValid(void)','  void  updateSensorDiag(float* diag)'},1,14);s.File11=reshape({ '  void  gpsInit(void)','  void  gpsParse(uint8_t* dataStream)','  void  updateStatus(uint8_t* completeMessage)','  void  updatePositionData(uint8_t* completeMessage)','  void  updateVelocityData(uint8_t* completeMessage)','  void  updateTimeData(uint8_t* completeMessage)','  void  getGpsMainData(float* data)','  uint32_t  CRC32Value(int32_t i)','  uint32_t  CalculateBlockCRC32(uint32_t ulCount, uint8_t *ucBuffer)','  uint16_t  charsToUint16(uint8_t* data)','  uint32_t  charsToUint32(uint8_t* data)','  float  charsToFloat(uint8_t* data)','  double  charsToDouble(uint8_t* data)'},1,13);s.File12=reshape({ '  void  getMidLevelCommands(float* commands)',' unsigned char  isApManual(uint16_t failsafe)','  float  getParamIdx(unsigned char idx)','  void  getRangeOfParams(uint8_t startIdx, uint8_t endIdx, float* parameters)','  float  getDynamic(void)','  void  getAttitude(float* attitude)','  void  getXYZ(float* xyz)','  void  getVned(float* xyz)','  uint8_t  getMaxWp(void)',' unsigned char  isWpFly(void)',' unsigned char  isPassthrough(void)','  void  setDiagnosticFloat(float * flValues)','  void  setDiagnosticShort(int16_t* shValues)','  void  getWP(unsigned char idx, float* WPpos)','  void  setLogFloat1(float * flValues)','  void  setLogFloat2(float * flValues)',' unsigned char  getApControlType(void)',' unsigned char  getPassValues(uint8_t* pasVals)','  void  setCurrentCommands(float airSpeed)','  void  getCurrentGPSPos(float* latLonAlt)','  void  setNavLong(float* values)','  void  setNavLat(float* values)','  void  setNavNav(float* values)','  void  getAccels(float * accels)','  void  getAccBias(float * bias)','  void  getRTB(uint8_t* rtb)','  void  getMobileLocation(float* loc)','  uint8_t  getNavMode(void)','  void  getISRLocation(float* loc)','  uint8_t  getISRCameraOption1(void)',' unsigned short  meanFilter5(unsigned short * values)','  uint8_t  justEnabled(uint8_t enableValue, uint8_t index)',' unsigned char  quickSort(unsigned short *arr, char elements)'},1,33);s.File13=reshape({ '  void  hilRead(unsigned char* hilChunk)','  void  hil_getRawRead(short * rawData)','  void  hil_getVned(float* vned)','  void  hil_getEuler(float* euler)','  void  hil_getRates(float* pqr)','  void  hil_getXYZ(float* xyz)',' unsigned int  hil_getTs(void)','  void  protDecodeHil(uint8_t* dataIn)'},1,8);s.File14=reshape({ '  void  cubeInit(void)','  void  getCubeData(short * cubeData)','  void  updateCubeData(void)','  int16_t  averageData(int16_t* theData, uint8_t count)',' unsigned short  write2Cube(unsigned short data2Send)','  void  __attribute__((interrupt, no_auto_psv)) _T5Interrupt(void)','  short  convert14BitToShort(short wordData)','  short  convert12BitToShort(short wordData)',' unsigned char  isCube16405(void)'},1,9);s.File15=reshape({ '  void  uartMavlinkBufferInit(void)','  uint16_t  PackHeartBeat(uint8_t system_id, uint8_t component_id)','  uint16_t  PackRawRC(uint8_t system_id, uint8_t component_id, mavlink_rc_channels_raw_t mlRC_Commands, uint32_t time_usec)','  uint16_t  PackVFR_HUD(uint8_t system_id, uint8_t component_id, mavlink_vfr_hud_t mlVfr_hud, uint32_t time_usec)','  uint16_t  PackRawIMU(uint8_t system_id, uint8_t component_id, mavlink_raw_imu_t mlRawIMUData ,uint32_t time_usec)','  char  sendQGCDebugMessage(const char * dbgMessage, char severity, unsigned char* bytesToAdd, char positionStart)','  uint16_t  PackGpsRawInt(uint8_t system_id, uint8_t component_id, mavlink_gps_raw_int_t mlRawGpsDataInt, uint32_t time_usec)','  uint16_t  PackGpsRawInt(uint8_t system_id, uint8_t component_id, mavlink_gps_raw_int_t mlRawGpsDataInt, uint32_t time_usec)','  uint16_t  PackScaledPressure(uint8_t system_id, uint8_t component_id, mavlink_scaled_pressure_t mlAirData, uint32_t time_usec)','  uint16_t  PackSysStatus(uint8_t system_id, uint8_t component_id, mavlink_sys_status_t mlSysStatus)'},1,10);"  ORDERING=None  SampleTime=-1  MCHP_MASTERLINK=|  PinDigitalInput=[]  PinDigitalOutput=[]  PinAnalogInput=[]
      | AUAV_V3_TestSensors_/Microchip Master
      | AUAV V3 Board
      | Busy Flag on D2 (RA6)
  Inner Loop/ Navigation : Subsystem
  LEDs_Driver : Subsystem  TreatAsAtomicUnit=on
      settings: RTWFileNameOpts=Use subsystem name
  MCU Load : MCHP_Blockset/Profiling/MCU Load  MCULoadPin=Dynamic Options  MCULoadPin_TXT=None  MCULoadMeasure=on  TIMER_Resolution=Dynamic Options  TIMER_Resolution_TXT="Resol: 0.9143(us)  -  Max: 59.9(ms)"  MCHP_TIMER_REQUEST={MCU_Load}{MCU_Load}21:5:0:0:[]:4194304;  MCHP_TIMER_RESULT=[3 65535 ]  MCHP_MASTERLINK=|  MCHP_COMPILED_INFO="CompiledSampleTime= [0.01   0 ];CompiledInportDataTypes=[ ];CompiledInportDataWidth=[];"  Info="Timer 3:  Resol: 914.2857143(ns)  -  Max: 59.9186(ms)"  SampleTime=.01
      | AUAV_V3_TestSensors/Microchip Master
      | AUAV V3 Board
      | Busy Flag on D2 (RA6)
  MPU_T : DataStoreMemory  DataStoreName=MPU_T  ReadBeforeWriteMsg=warning  WriteAfterWriteMsg=warning  WriteAfterReadMsg=warning  OutDataTypeStr=uint16
      settings: RTWStateStorageClass=ExportedGlobal
  Mavlink_TX_Adapter : Subsystem  TreatAsAtomicUnit=on
      settings: RTWFileNameOpts=Use subsystem name
  Microchip Master AUAV V3 Board Busy Flag on D2 (RA6) : MCHP_Blockset/System Configuration/Microchip Master  Priority=1  PICREF=33EP512MU810  TIMESTEP_REF="Timer  ( 0.01s + [-0.0045714%] ==> 0.0099995s )"  BUSYFLAG=Dynamic Options  BUSYFLAG_TXT=A6 / Pin[91]  PWRTEN=PWRT enabled  BOREN=Disable  BODENV=2.7V  BORV=Brown-out Reset set at 2.0V  FPWRT=128ms  DSBOREN=Deep Sleep BOR enabled in Deep Sleep  DSLPBOR=Deep Sleep BOR enabled in Deep Sleep  MCLRE=Enabled  PMDL1WAY=Allow only one reconfiguration  RSTPRI=Device will obtain reset instruction from Primary flash  TEMP=Not used  SOSCSRC=Analog Mode for use with crystal  SOSCSEL=Secondary oscillator configured for high-power operation  IOL1WAY=Allow only one reconfiguration  ALTVREF=Voltage reference input; ADC =RA9/RA10 Comparator =RA9;RA10  DISUVREG=Regulator is disabled  DSSWEN=Deep Sleep is controlled by the register bit DSEN  LPCFG=Disabled - regardless of RETEN  RTCBAT=RTC operation is continued through VBAT  VBTBOR=VBAT BOR enabled  WUTSEL=Default regulator start-up time used  POWERSAVE=off  FNOSC=Primary oscillator (XT; HS; EC)  FPR=ECIO w/ PLL 16x  FOSFPR=HS3 w/PLL 16x  FOS=Internal Fast RC  FRANGE=High Range  OSCILLATOR_SELECT=Crystal / Ceramic resonator  OSCILLATOR_SELECT_spd=Crystal / Ceramic resonator  QUARTZ=8e6  QUARTZ_spd=8e6  ACTIV_PLL=on  ACTIV_PLL_spd=on  MIPS_DESIRED=70e6  MIPS_DESIRED_spd=70e6  FPLLMUL=24x Multiplier  FPLLIDIV=8x Divider  POSCFREQ=Primary oscillator/external clock input frequency greater than 8MHz  POSCMD=XT Crystal Oscillator Mode  POSCMOD=Primary Oscillator Disabled  MIPS=70 * 1e6  FPLLODIV=32x Divider  PLLKEN=Clock switch to PLL source will wait until the PLL lock signal is valid.  FCKSM=Both Clock Switching and Fail-safe Clock Monitor are enabled  FCKSMEN=Sw Disabled; Mon Disabled  IESO=Start up with FRC; then switch  DSWDTPS=1:2;147;483;648 (25.7 Days)  FWDTEN=Disable  FWDTWINSZ=Window Size is 25%  FWPSA=1:512  FWPSA0=1:128  FWPSB=1:16  WDT=Disable  WDTPOST=1:32768  WDTPRE=1:128  WDTPS=1:32768  WINDIS=Watchdog Timer in Non-Window mode  WWDTEN=Non-Window mode  DSWDTEN=DSWDT enabled  DSWDTOSC=DSWDT uses Low Power RC Oscillator (LPRC)  FPBDIV=Pb_Clk is Sys_Clk/8  FSOSCEN=Enable SOSC  LPRCSEL=High Power; High Accuracy Mode  OSCIOFCN=OSCO/CLKO/RC15 functions as CLKO (FOSC/2)  OSCIOFNC=OSC2 is general purpose digital I/O pin  LVRCFG=Low Voltage regulator is not available  PLL_96MHZ=Enabled  PLL96MHZ=96 MHz PLL Startup is enabled automatically on start-up  PLLDIV=PLL is disabled  WDTCLK=WDT uses LPRC  WDTCMX=WDT clock source is determined by the WDTCLK Configuration bits  WDTWIN=WDT Window is 25% of WDT period  APL=Aux Flash Code protect is disabled  APLK=Aux Flash Write Protection and Code Protection is Disabled  AWRP=Auxiliary program memory is not write-protected  BSS=No boot program Flash segment  BWP=Protection Disabled  BWRP=Boot Segment may be written  CP=Protection Disabled  EBS=No Boot EEPROM  ESS=No Segment Data EEPROM  GCP=Disable  GSS=General Segment Code protect is disabled  GSS0=No protection  GSSK=General Segment Write Protection and Code Protection is Disabled  GWRP=General Segment may be written  PWP=Disable  RBS=No Boot RAM  RSS=No Secure RAM  SSS=No Secure Segment  SWRP=Secure segment may be written  WPCFG=Disable  WPDIS=Disable  WPEND=Write Protect from WPFP to the last page of memory  WPFP=Page 127 (0x1FC00)  ICESEL=Communicate on PGEC1/PGED1  ICS=Communicate on PGEC3 and PGED3  JTAGEN=Disable  COE=Reset Into Operational Mode  RES=Not used  DEBUG=Debugger is Disabled  BACKBUG=Not used  BKBUG=Device resets into Operational mode  ALTI2C=I2C mapped to SDA1/SCL1 pins  ALTI2C1=SDA1/SCK1 pins are selected as the I/O pins for I2C1  ALTI2C2=ASDA2/ASCK2 pins are selected as the I/O pins for I2C2  ALTQIO=QEA1; QEB1; INDX1 are selected as inputs to QEI1  ALTSS1=SS1A is selected as the I/O pin for SPI1  CMPPOL0=Hysteresis is applied to falling edge  CMPPOL1=Hysteresis is applied to falling edge  FCANIO=Default CAN I/O  FETHIO=Default Ethernet I/O  FMIIEN=MII Enabled  FSRSSEL=SRS Priority 7  FUSBIDIO=Controlled by the USB Module  FVBUSONIO=Controlled by USB Module  HPOL=Active High  HYST0=45 mV Hysteresis  HYST1=45 mV Hysteresis  I2C1SEL=Use Default SCL1/SDA1 Pins For I2C1  LPOL=Active High  PWMPIN=Control with PORT/TRIS regs  RTCOSC=RTCC uses Secondary Oscillator (SOSC)  UPLLEN=USB PLL is enabled  UPLLIDIV=12x Divider  ATMOD8=Not used  ALTPMP=EPMP pins are in default location mode  I2C2SEL=I2C2 is multiplexed to SDA2/RA3 and SCL2/RA2  ALTADREF=AVREF+/AVREF- are mapped to RA9/RA10  ALTCVREF=CVREF+/CVREF- are mapped to RA9/RA10  PWMLOCK=PWM registers may be written without key sequence  MCHP_TIMER_REQUEST={Time Step}{TS}0:2:3:1:[]:700000;  MCHP_TIMER_RESULT=[2 10936.499999999987 ]  MCHP_PORT={Busy Flag}{Busy}0:1:A6;  MCHP_PLLRegisters="[5    243  16385     -1]"  MCHPVAR="MCHP.id = '33EP512MU810';MCHP.idN = [33  512  810];MCHP.idL = {'EP','MU',''};MCHP.Arch =3;MCHP.Rx = reshape([17   25   -1   72   93   87   90   -1   -1   -1   -1   38   24    6   76   94   88   89   -1   -1   -1   -1   58   23    7   77   98   52   57   -1   -1   -1   -1   59   22    8   78   99   51   56   -1   -1   -1   -1   60   21    9   81  100   49   -1   -1   -1   -1   -1   61   20   -1   82    3   50   -1   -1   -1   -1   -1   91   26   -1   83    4   -1   10   -1   -1   -1   -1   92   27   -1   84    5   -1   11   -1   -1   -1   -1   -1   32   -1   68   18   53   12   -1   -1   -1   -1   28   33   -1   69   19   -1   14   -1   -1   -1   -1   29   34   -1   70   -1   -1   -1   -1   -1   -1   -1   -1   35   -1   71   -1   -1   -1   -1   -1   -1   -1   -1   41   63   79   -1   40   96   -1   -1   -1   -1   -1   42   73   80   -1   39   97   -1   -1   -1   -1   66   43   74   47   -1   -1   95   -1   -1   -1   -1   67   44   64   48   -1   -1    1   -1   -1   -1   -1],11,16);MCHP.RP = [-1   -1   -1   -1   -1   -1   -1   -1   -1   -1   -1   -1   -1   -1   -1   -1   -1   -1   -1   -1   -1   -1   -1   -1   -1   -1   -1   -1   -1   -1   -1   -1   -1   -1   -1   -1   -1   -1   -1   -1   -1   -1   -1   -1   -1   -1   -1   -1   -1   -1   -1   -1   -1   -1   -1   -1   -1   -1   -1   -1   -1   -1   -1   -1   48   49   50   51   52   53   54   55   -1   -1   -1   -1   -1   -1   -1   63   64   -1   66   -1   68   69   -1   71   -1   -1   -1   -1   -1   -1   -1   -1   80   81   82   83   84   85   -1   -1   88   -1   -1   -1   92   93   -1   -1   96   97   -1   -1   -1   -1  102   -1  104   -1   -1   -1   -1  109  110  111];MCHP.RPI = [-1   -1   -1   -1   -1   -1   -1   -1   -1   -1   -1   -1   -1   -1   -1   -1    0    1    2    3    4    5    6    7   -1   -1   -1   -1   -1   -1   14   15   16   17   18   19   20   21   22   23   24   25   26   27   28   29   30   31   -1   33   34   35   36   -1   -1   -1   -1   -1   -1   -1   44   45   46   -1   -1   -1   -1   -1   -1   -1   -1   -1   56   57   58   59   60   61   62   -1   -1   65   -1   67   -1   -1   70   -1   72   73   -1   -1   -1   -1   -1   -1   -1   -1   -1   -1   -1   -1   -1   -1   -1   -1   -1   -1   -1   -1   -1   -1   -1   -1   -1   -1   -1   -1   -1  103   -1  105   -1   -1  108];MCHP.PPS.reg_RPINRx = [-1  1  1  1  1 -1  1  1  1  1  1  1  1  1  1  1  1  1  1  1  1  1 -1 -1  1  1  1  1  1  1  1  1  1  1  1  1  1  1  1  1  1  1  1 -1 -1 -1  1 -1 -1 -1 -1 -1  1  1  1  1  1  1  1  1  1 -1  1  1  1 -1  1  1  1  1  1  1  1  1 -1  1  1  1  1  1  1  1  1 -1  1  1  1];MCHP.RPINR_list = {'1','INT1','INT2','INT3','INT4','T1CK','T2CK','T3CK','T4CK','T5CK','T6CK','T7CK','T8CK','T9CK','IC1','IC2','IC3','IC4','IC5','IC6','IC7','IC8','OCFA','OCFB','FLT1','FLT2','FLT3','FLT4','QEA1','QEB1','INDX1','HOME1','QEA2','QEB2','INDX2','HOME2','U1RX','U1CTS','U2RX','U2CTS','SDI1','SCK1','SS1','44','SDI2','SCK2','SS2','48','CSDIR','CSCK','COFSIN','52','C1RX','C2RX','U3RX','U3CTS','U4RX','U4CTS','SDI3','SCK3','SS3','62','SDI4','SCK4','SS4','66','IC9','IC10','IC11','IC12','IC13','IC14','IC15','IC16','OCFC','SYNCI1','SYNCI2','DTCMP1','DTCMP2','DTCMP3','DTCMP4','DTCMP5','DTCMP6','DTCMP7','FLT5','FLT6','FLT7','88','89','SENT1','SENT2','92'};MCHP.RPOR_list = {'1','U1TX','U1RTS','U2TX','U2RTS','SDO1','SCK1','SS1','SDO2','SCK2','SS2','CSDO','CSCK','COFS','C1TX','C2TX','OC1','OC2','OC3','OC4','OC5','OC6','OC7','OC8','C1OUT','C2OUT','C3OUT','U3TX','U3RTS','U4TX','U4RTS','SDO3','SCK3','SS3','SDO4','SCK4','SS4','OC9','OC10','OC11','OC12','OC13','OC14','OC15','OC16','SYNCO1','SYNCO2','QEI1CCMP','QEI2CCMP','REFCLK','C4OUT'};MCHP.PPS.map_RPnR_RPORx = [64   65   66   67   68   69   70   71   79   80   82   84   85   87   96   97   98   99  100  101   -1   -1  104  108  109  112  113  118  120  125  126  127];MCHP.memory.RAM = [53248];MCHP.memory.RAM_XBegin = [4096];MCHP.memory.RAM_YBegin = [36864];MCHP.memory.RAM_dma = [53248];MCHP.fcy.periph = 70000000;MCHP.TimeStepFactor = [0.99995];MCHP.fcy.MIPS = 70000000;MCHP.TimeStep_Timer = 2;MCHP.NTIMERS = 9;MCHP.PowerSave = [0];MCHP.DMA.Num = [15];MCHP.DMA.CNTmax = [16383];MCHP.QEI.QEICONx = [49023  49023     -1     -1     -1     -1];MCHP.QEI.QEItype = [2];MCHP.QEI.Port_QEI_INDX = [-1 -1];MCHP.QEI.Port_QEI_QEA = [-1 -1];MCHP.QEI.Port_QEI_QEB = [-1 -1];MCHP.QEI.Port_QEI_UPDN = [-1 -1];MCHP.ADC.ADCONx = [47103  59391  40959    263      0      0];MCHP.ADC.ADCHS_0 = [40863   1799];MCHP.ADC.ANtype = [3  1];MCHP.ADC.Flags = [1  0];MCHP.ADC.Buffer = [16  16];MCHP.ADC.port = [16  17  18  19  20  21  22  23  24  25  26  27  28  29  30  31  33  34  35  36  72  73   6   7  64  65  66  67  68  69  70  71  -1  -1  -1  -1  -1  -1  -1  -1  -1  -1  -1  -1  -1  -1  -1  -1  -1  -1  -1  -1  -1  -1  -1  -1  -1];MCHP.ADC.port_VrefP = [-1];MCHP.ADC.port_VrefM = [-1];MCHP.ADC.port_AVdd = [-1];MCHP.ADC.port_AVss = [-1];MCHP.PWM_HS.Flags = [6  2  1];MCHP.PWM.port_FLT = [-1 -1 -1 -1 -1 -1 -1 -1 -1 -1 -1 -1 -1 -1 -1 -1 -1 -1 -1 -1 -1 -1 -1 -1 -1 -1 -1 -1 -1 -1 -1 -1 -1];MCHP.PWM.PWMRef = -1;MCHP.PWM.Flag = 0;MCHP.PWM.Port_PWM_l = [64  66  68  70  33  35  -1  -1  -1;-1 -1 -1 -1 -1 -1 -1 -1 -1];MCHP.PWM.Port_PWM_h = [65  67  69  71  34  36  -1  -1  -1;-1 -1 -1 -1 -1 -1 -1 -1 -1];MCHP.IC.Port = [32767  32767  32767  32767  32767  32767  32767  32767  32767  32767  32767  32767  32767  32767  32767  32767];MCHP.IC.type = 1;MCHP.OC.Port = [32767  32767  32767  32767  32767  32767  32767  32767  32767  32767  32767  32767  32767  32767  32767  32767];MCHP.OC.type = 1;MCHP.CN.Port = [-1 -1 -1 -1 -1 -1 -1 -1 -1 -1 -1 -1 -1 -1 -1 -1 -1 -1 -1 -1 -1 -1 -1 -1 -1 -1 -1 -1 -1 -1 -1 -1 -1 -1 -1 -1 -1 -1 -1 -1 -1 -1 -1 -1 -1 -1 -1 -1 -1 -1 -1 -1 -1 -1 -1 -1 -1 -1 -1 -1 -1 -1 -1 -1 -1 -1 -1 -1 -1 -1 -1 -1 -1 -1 -1 -1 -1 -1 -1 -1 -1 -1 -1 -1 -1];MCHP.CN.PullUp = [50943  65535  61470  65535   1023  12607  62403      0      0      0      0];MCHP.CN.type = 1;MCHP.CN.Flag_PullDown = 1;MCHP.SPI.Refs = [1  2  3  4  0  0];MCHP.SPI.SPIxCON1 = 8191;MCHP.SPI.SPIxCON2 = 57347;MCHP.SPI.Port_SDI = [-1  103   -1   -1   -1   -1];MCHP.SPI.Port_SDO = [-1  104   -1   -1   -1   -1];MCHP.SPI.Port_SCK = [-1  102   -1   -1   -1   -1];MCHP.SPI.Port_SS = [-1 -1 -1 -1 -1 -1];MCHP.I2C.Refs = [1  2  0  0  0];MCHP.I2C.I2CxCON = 49151;MCHP.I2C.NewRegName = 1;MCHP.I2C.Port_SDA = [-1  84  -1  -1  -1];MCHP.I2C.Port_SCL = [-1  85  -1  -1  -1];MCHP.I2C.Port_ASDA = [57   3  -1  -1  -1];MCHP.I2C.Port_ASCL = [58   2  -1  -1  -1];MCHP.I2C.Fuse_Port_SCL_SDA = [17  18  -1  -1  -1;1  1 -1 -1 -1];MCHP.I2C.Fuse_Port_ASCL_ASDA = [17  18  -1  -1  -1;2  2 -1 -1 -1];MCHP.Comp.Port_CVrefin = [-1];MCHP.Comp.Port_CVref = [26];MCHP.Comp.Port_CVref1O = [-1];MCHP.Comp.Port_CVref2O = [-1];MCHP.Comp.Port_CxOUT = [32767  32767  32767     -1     -1];MCHP.Comp.Port_OAxOUT = [-1 -1 -1 -1 -1];MCHP.Comp.Port_CxINP = [21  19  55  -1  -1];MCHP.Comp.Port_CxINM = [103   20  102   -1;105   18  104   -1;46  54  45  -1;-1 -1 -1 -1;-1 -1 -1 -1];MCHP.Comp.nComp = [3  0  0];MCHP.Comp.OpAmp = [0];MCHP.Comp.CVRCON = [2047     0];MCHP.UART.port_Rx = [32767  32767  32767  32767     -1     -1];MCHP.UART.port_Tx = [32767  32767  32767  32767     -1     -1];MCHP.UART.port_ARx = [-1 -1];MCHP.UART.port_ATx = [-1 -1];MCHP.UART.port_RTS = [32767  32767  32767  32767     -1     -1];MCHP.UART.port_CTS = [32767  32767  32767  32767     -1     -1];MCHP.UART.reg_UxMODE = [48127  48127  48127  48127     -1     -1];MCHP.UART.reg_UxSTA = [61439  61439  61439  61439     -1     -1];"  MCHP_CRC=3107746  BTMODE=Device is in Single Boot (legacy) mode  RES1=Not used  PLLSS=PLL is fed by the Primary oscillator  RES2=Not used  ALTCMPI=C1INC is on RB13; C2INC is on RB9 and C3INC is on RA0  BOREN1=BOR Enabled [When BOREN=1]  ALTRB6=Append the RP6/ASCL1/PMPD6 functions of RB6 to RA1 pin functions  RETCFG=Retention regulator is not available  DFMCY=Not used  BSS2=No Boot Segment  CWRP=Configuration Segment may be written  CSS=No Protection (other than CWRP)  AIVTDIS=Disabled AIVT  BSLIM=Not used  WDTEN=Disable  BTSWP=Not used  DBCC=Not used  CTXT1=Not Assigned  CTXT2=Not Assigned  SEQNUM=Not used  nSEQNUM=Not used  BOREN0=Enabled  DMTIVT=Not used  DMTCNT=2^31 (2147483648)  DMTEN=Dead Man Timer is Enabled and cannot be disabled by software  ON=Not used  USERID=Not used  RESERVED1=Not used  PGL1WAY=Allow only one reconfiguration  FPLLRNG=34-68 MHz Input  FPLLICLK=FRC is input to the System PLL  FPLLMULT=PLL Multiply by 128  UPLLFSEL=USB PLL input is 24 MHz  DMTINTV=Window/Interval value is 127/128 counter value  WDTSPGM=WDT stops during Flash programming  FDMTEN=Deadman Timer is disabled  TRCEN=Trace features in the CPU are enabled  BOOTISA=Boot code and Exception code is MIPS32  FECCCON=ECC and Dynamic ECC are disabled (ECCCON bits are writable)  FSLEEP=Flash is powered down when the device is in Sleep mode  DBGPER=Allow CPU access to all permission regions  EJTAGBEN=Normal EJTAG functionality  TSEQ=Not used  CSEQ=Not used
  Model Info : simulink/Model-Wide Utilities/Model Info  Frame=on  DisplayStringWithTags=|  HorizontalTextAlignment=Center  LeftAlignmentValue=0.5  SourceBlockDiagram=AUAV_V3_TestSensors_Cmp  TagMaxNumber=20
      | %<Description>
      | %<ModifiedBy>
      | %<ModelVersion>
      | %<LastModifiedBy>
  Mux : Mux  Inputs=2
  PAR_L1_OMEGA PAR_L1_M PAR_L1_GAMMA PAR_L1_ON_OFF : DataStoreRead  DialogController=Simulink.DDGSource  DataStoreName=mlParamInterface  DataStoreElements=mlParamInterface.param(22)#mlParamInterface.param(23)#mlParamInterface.param(24)#mlParamInterface.param(25)
  PAR_NAV_ISR_FAC PAR_PID_RMIX_ON PAR_PID_RMIX_P : DataStoreRead  DialogController=Simulink.DDGSource  DataStoreName=mlParamInterface  DataStoreElements=mlParamInterface.param(26)#mlParamInterface.param(27)#mlParamInterface.param(28)
  PAR_NAV_L2_BASE PAR_NAV_PRETURN_K PAR_NAV_SSCOMP_ON : DataStoreRead  DialogController=Simulink.DDGSource  DataStoreName=mlParamInterface  DataStoreElements=mlParamInterface.param(19)#mlParamInterface.param(20)#mlParamInterface.param(21)
  PID Gains [updated 4.28.16] : Subsystem
  Passthrough Logic : Subsystem
  Pilot : simulink/Sources/Counter Limited  Commented=on  uplimit=1  tsamp=1.0
  Pilot LED and HIL Control Pins : Subsystem  Commented=on
  Port Info : MCHP_Blockset/System Info/Port Info  MCHP_MASTERLINK=|
      | AUAV_V3_TestSensors/Microchip Master
      | AUAV V3 Board
      | Busy Flag on D2 (RA6)
  Position_and_Attitude_Filter : Subsystem  TreatAsAtomicUnit=on
      settings: RTWFileNameOpts=Use subsystem name
  RC_Driver : Subsystem  Commented=on  TreatAsAtomicUnit=on
  Sensor_Data_Adapter : Subsystem  TreatAsAtomicUnit=on
      settings: RTWFileNameOpts=Use subsystem name
  Servo In Out : Subsystem  Commented=on
  Terminator : Terminator  Commented=on
  Terminator1 : Terminator  Commented=on
  Terminator2 : Terminator  Commented=on
  Terminator{4..8} (5 alike) : Terminator
  TimeSinceBoot_usec : DataStoreMemory  DataStoreName=time_since_boot_usec  ReadBeforeWriteMsg=warning  WriteAfterWriteMsg=warning  WriteAfterReadMsg=warning  OutDataTypeStr=uint32
  Timer Info : MCHP_Blockset/System Info/Timer Info  MCHP_MASTERLINK=|
      | AUAV_V3_TestSensors/Microchip Master
      | AUAV V3 Board
      | Busy Flag on D2 (RA6)
  To Control MCU : Subsystem
  Trim Vals [updated 4.28.16] : Subsystem
  UART Configuration UAV V3 UART 3 : MCHP_Blockset/BUS UART/UART Configuration  UART_REF=1  BAUD_Choice=Dynamic Options  BAUD_Choice_TXT="57600         [-0.06%]"  BAUD_Choice_IR=Dynamic Options  BAUD_Choice_IR_TXT=[]  BAUD_Custom=115200  IRDA=off  ALT_IO=on  PIN_RX=Dynamic Options  PIN_RX_TXT=F2 / P98 / Pin[52]  PIN_TX=Dynamic Options  PIN_TX_TXT=F3 / P99 / Pin[51]  FlowControl=None  PIN_CTS=Dynamic Options  PIN_CTS_TXT=A0 / P16 / Pin[17]  PIN_RTS=Dynamic Options  PIN_RTS_TXT=D0 / P64 / Pin[72]  MCHP_PORT="{UART1  Tx}{U1TX}3:1:P99;"  MCHP_MASTERLINK=|  MCHP_COM_ExtPil=off  TX_IMPLEMENTATION=Circular Buffer  TX_INT_PRIORITY=1  TX_INT_WHEN=is empty & last char is sent  TX_CIRCULAR_SIZE=512  TX_DMA_CHANNEL="0   (Lowest Priority)"  TX_DMA_SIZE=[]  RX_IMPLEMENTATION=Do not implement Rx  RX_INT_PRIORITY=1  RX_INT_WHEN=receive 1 character  RX_CIRCULAR_SIZE=128  InitSequence_chkbox=on  BAUD_Choice_InitSeq=Dynamic Options  BAUD_Choice_InitSeq_TXT="110         [-0.00%]"  BAUD_Choice_IR_InitSeq=Dynamic Options  BAUD_Choice_IR_InitSeq_TXT=0  BAUD_Custom_InitSeq=0  InitSequence='Hello World'
      | AUAV_V3_TestSensors/Microchip Master
      | AUAV V3 Board
      | Busy Flag on D2 (RA6)
  UART Configuration UAV V3 UART 4 GPS : MCHP_Blockset/BUS UART/UART Configuration  UART_REF=4  BAUD_Choice=Dynamic Options  BAUD_Choice_TXT="38400         [-0.06%]"  BAUD_Choice_IR=Dynamic Options  BAUD_Choice_IR_TXT=[]  BAUD_Custom=115200  IRDA=off  ALT_IO=on  PIN_RX=Dynamic Options  PIN_RX_TXT=E6 / P86 / Pin[4]  PIN_TX=Dynamic Options  PIN_TX_TXT=E5 / P85 / Pin[3]  FlowControl=None  PIN_CTS=Dynamic Options  PIN_CTS_TXT=A0 / P16 / Pin[17]  PIN_RTS=Dynamic Options  PIN_RTS_TXT=D0 / P64 / Pin[72]  MCHP_PORT="{UART4  Tx}{U4TX}3:1:P85;"  MCHP_MASTERLINK=|  MCHP_COM_ExtPil=off  TX_IMPLEMENTATION=Circular Buffer  TX_INT_PRIORITY=1  TX_INT_WHEN=is empty & last char is sent  TX_CIRCULAR_SIZE=512  TX_DMA_CHANNEL="0   (Lowest Priority)"  TX_DMA_SIZE=[]  RX_IMPLEMENTATION=Do not implement Rx  RX_INT_PRIORITY=1  RX_INT_WHEN=receive 1 character  RX_CIRCULAR_SIZE=128  InitSequence_chkbox=on  BAUD_Choice_InitSeq=Dynamic Options  BAUD_Choice_InitSeq_TXT="110         [-0.00%]"  BAUD_Choice_IR_InitSeq=Dynamic Options  BAUD_Choice_IR_InitSeq_TXT=0  BAUD_Custom_InitSeq=0  InitSequence='Hello World'
      | AUAV_V3_TestSensors/Microchip Master
      | AUAV V3 Board
      | Busy Flag on D2 (RA6)
  Update PWM Commands and Send Telemetry [updated 4.27.16] : Subsystem
  Update SysStatus Load : DataStoreWrite  DataStoreName=mlSysStatus  DataStoreElements=mlSysStatus.load
  Update time : DataStoreWrite  DialogController=Simulink.DDGSource  DataStoreName=time_since_boot_usec  DataStoreElements=time_since_boot_usec
  get Nav Vars [updated 4.28.16] : Subsystem
  isPassthrough : DataStoreRead  DialogController=Simulink.DDGSource  DataStoreName=mlHeartbeatLocal  DataStoreElements=mlHeartbeatLocal.custom_mode
  isWpFly? : DataStoreRead  DialogController=Simulink.DDGSource  DataStoreName=mlHeartbeatLocal  DataStoreElements=mlHeartbeatLocal.custom_mode
  mlAirData : DataStoreMemory  DataStoreName=mlAirData  ReadBeforeWriteMsg=warning  WriteAfterWriteMsg=warning  WriteAfterReadMsg=warning  OutDataTypeStr=Bus: mavlink_scaled_pressure_t
      settings: RTWStateStorageClass=ExportedGlobal
  mlAttitudeData : DataStoreMemory  DataStoreName=mlAttitudeData  ReadBeforeWriteMsg=warning  WriteAfterWriteMsg=warning  WriteAfterReadMsg=warning  OutDataTypeStr=Bus: mavlink_attitude_t
      settings: RTWStateStorageClass=ExportedGlobal  LockScale=on
  mlAttitudeData1 : DataStoreMemory  DataStoreName=mlAttitudeSol  ReadBeforeWriteMsg=warning  WriteAfterWriteMsg=warning  WriteAfterReadMsg=warning  OutDataTypeStr=Bus: mavlink_attitude_t
      settings: RTWStateStorageClass=ExportedGlobal  LockScale=on
  mlGSLocationFloat : DataStoreMemory  DataStoreName=mlGSLocationFloat  ReadBeforeWriteMsg=warning  WriteAfterWriteMsg=warning  WriteAfterReadMsg=warning  OutDataTypeStr=Bus: mavlink_coordinate_float_t
      settings: RTWStateStorageClass=ExportedGlobal
  mlGpsData : DataStoreMemory  DataStoreName=mlGpsData  ReadBeforeWriteMsg=warning  WriteAfterWriteMsg=warning  WriteAfterReadMsg=warning  OutDataTypeStr=Bus: mavlink_gps_raw_int_t
      settings: RTWStateStorageClass=ExportedGlobal
  mlHeartbeatLocal : DataStoreMemory  DataStoreName=mlHeartbeatLocal  ReadBeforeWriteMsg=warning  WriteAfterWriteMsg=warning  WriteAfterReadMsg=warning  OutDataTypeStr=Bus: mavlink_heartbeat_t
      settings: RTWStateStorageClass=ExportedGlobal
  mlISR : DataStoreMemory  DataStoreName=mlISR  ReadBeforeWriteMsg=warning  WriteAfterWriteMsg=warning  WriteAfterReadMsg=warning  OutDataTypeStr=Bus: mavlink_isr_location_t
      settings: RTWStateStorageClass=ExportedGlobal
  mlLocalPositionData : DataStoreMemory  DataStoreName=mlLocalPositionData  ReadBeforeWriteMsg=warning  WriteAfterWriteMsg=warning  WriteAfterReadMsg=warning  OutDataTypeStr=Bus: mavlink_local_position_ned_t
      settings: RTWStateStorageClass=ExportedGlobal
  mlMidLevelCommands : DataStoreMemory  DataStoreName=mlMidLevelCommands  ReadBeforeWriteMsg=warning  WriteAfterWriteMsg=warning  WriteAfterReadMsg=warning  OutDataTypeStr=Bus: mavlink_mid_lvl_cmds_t
      settings: RTWStateStorageClass=ExportedGlobal
  mlMobileLocation : DataStoreMemory  DataStoreName=mlMobileLocation  ReadBeforeWriteMsg=warning  WriteAfterWriteMsg=warning  WriteAfterReadMsg=warning  OutDataTypeStr=Bus: mavlink_slugs_mobile_location_t
      settings: RTWStateStorageClass=ExportedGlobal
  mlNavigation : DataStoreMemory  DataStoreName=mlNavigation  ReadBeforeWriteMsg=warning  WriteAfterWriteMsg=warning  WriteAfterReadMsg=warning  OutDataTypeStr=Bus: mavlink_slugs_navigation_t
      settings: RTWStateStorageClass=ExportedGlobal
  mlParamINterface : DataStoreMemory  DataStoreName=mlParamInterface  ReadBeforeWriteMsg=warning  WriteAfterWriteMsg=warning  WriteAfterReadMsg=warning  OutDataTypeStr=Bus: pi_struct
      settings: RTWStateStorageClass=ExportedGlobal
  mlPilotConsoleData : DataStoreMemory  DataStoreName=mlPilotConsoleData  ReadBeforeWriteMsg=warning  WriteAfterWriteMsg=warning  WriteAfterReadMsg=warning  OutDataTypeStr=Bus: mavlink_rc_channels_raw_t
      settings: RTWStateStorageClass=ExportedGlobal
  mlRawImuData : DataStoreMemory  DataStoreName=mlRawImuData  ReadBeforeWriteMsg=warning  WriteAfterWriteMsg=warning  WriteAfterReadMsg=warning  OutDataTypeStr=Bus:mavlink_raw_imu_t
      settings: RTWStateStorageClass=ExportedGlobal
  mlRawPressureData : DataStoreMemory  DataStoreName=mlRawPressureData  ReadBeforeWriteMsg=warning  WriteAfterWriteMsg=warning  WriteAfterReadMsg=warning  OutDataTypeStr=Bus: mavlink_raw_pressure_t
      settings: RTWStateStorageClass=ExportedGlobal
  mlRawServo : DataStoreMemory  DataStoreName=mlPwmCommands  ReadBeforeWriteMsg=warning  WriteAfterWriteMsg=warning  WriteAfterReadMsg=warning  OutDataTypeStr=Bus: mavlink_servo_output_raw_t
      settings: RTWStateStorageClass=ExportedGlobal
  mlSysStatus : DataStoreMemory  DataStoreName=mlSysStatus  ReadBeforeWriteMsg=warning  WriteAfterWriteMsg=warning  WriteAfterReadMsg=warning  OutDataTypeStr=Bus: mavlink_sys_status_t
      settings: RTWStateStorageClass=ExportedGlobal
  mlVISensor : DataStoreMemory  DataStoreName=mlVISensor  ReadBeforeWriteMsg=warning  WriteAfterWriteMsg=warning  WriteAfterReadMsg=warning  OutDataTypeStr=Bus: mavlink_volt_sensor_t
      settings: RTWStateStorageClass=ExportedGlobal  LockScale=on
  mlVfr_hud : DataStoreMemory  DataStoreName=mlVfr_hud  ReadBeforeWriteMsg=warning  WriteAfterWriteMsg=warning  WriteAfterReadMsg=warning  OutDataTypeStr=Bus: mavlink_vfr_hud_t
      settings: RTWStateStorageClass=ExportedGlobal
  mlWpValues : DataStoreMemory  DataStoreName=mlWpValues  ReadBeforeWriteMsg=warning  WriteAfterWriteMsg=warning  WriteAfterReadMsg=warning  OutDataTypeStr=Bus: mavlink_mission_item_values_t
      settings: RTWStateStorageClass=ExportedGlobal
  myMux Fun1 : MATLAB Function  TreatAsAtomicUnit=on
  myMux Fun2 : MATLAB Function  TreatAsAtomicUnit=on
  myMux Fun3 : MATLAB Function  TreatAsAtomicUnit=on
  myMux Fun4 : MATLAB Function  TreatAsAtomicUnit=on
  myMux Fun5 : MATLAB Function  TreatAsAtomicUnit=on
  tag scope: HILON=global, HIL_FLAG=global
  wires:
  Counter Free-Running/1 -> Gain/1
  Gain/1 -> Data Type Conversion6/1
  Data Type Conversion6/1 -> Update time/1
  MCU Load/1 -> Update SysStatus Load/1  "U3 CH4"
  RC_Driver/1(Out1) -> Terminator/1
  RC_Driver/3(Out3) -> Terminator2/1
  RC_Driver/2(Out2) -> Terminator1/1
  Control Surface Input/1(Pilot Console) -> Goto21/1
  Sensor_Data_Adapter/2(Accel (m/s^2)) -> [Accel]
  Sensor_Data_Adapter/1(Omega (rad/s)) -> [Omega]
  Sensor_Data_Adapter/3(Mag (mG)) -> [Mag]
  Sensor_Data_Adapter/4(Baro Alt (m)) -> [BaroAlt]
  Sensor_Data_Adapter/6(GPS) -> [GPSMain]
  [Omega] -> Position_and_Attitude_Filter/2(Omega (rad/s))
  [Accel] -> Position_and_Attitude_Filter/1(A_sens(m/s^2))
  Position_and_Attitude_Filter/1(euler_hat (rad)) -> myMux Fun2/1(u1)
  [GPSMain] -> Position_and_Attitude_Filter/3(GPSMain)
  [BaroAlt] -> Position_and_Attitude_Filter/4(Baro Alt (m))
  myMux Fun2/1(y) -> [Attitude]
  myMux Fun3/1(y) -> [Position]
  myMux Fun4/1(y) -> [Biases]
  Position_and_Attitude_Filter/3(Pxyz_hat (m)) -> [Pos_Hat], myMux Fun3/1(u1)
  Position_and_Attitude_Filter/4(Vned_hat (m/s)) -> [Vned], myMux Fun3/2(u2)
  Position_and_Attitude_Filter/2(pqr_hat (rad/s)) -> myMux Fun2/2(u2)
  Position_and_Attitude_Filter/5(GyroBias (rad/s)) -> myMux Fun4/1(u1)
  Position_and_Attitude_Filter/6(Accel Bias (m/s)) -> [Accel_Bias], myMux Fun4/2(u2)
  Pilot/1 -> Pilot LED and HIL Control Pins/1(In1)  "1Hz"
  Trim Vals [updated 4.28.16]/4(dE Trim) -> Inner Loop/ Navigation/7(dE Trim (rad))
  Trim Vals [updated 4.28.16]/1(dT Trim) -> Inner Loop/ Navigation/4(dTTrim (abs))
  Trim Vals [updated 4.28.16]/2(dA Trim) -> Inner Loop/ Navigation/5(dA Trim (rad))
  Trim Vals [updated 4.28.16]/3(dR Trim) -> Inner Loop/ Navigation/6(dRTrim (rad))
  PID Gains [updated 4.28.16]/1(uHold PID) -> Inner Loop/ Navigation/8(U_hold PID)
  PID Gains [updated 4.28.16]/2(he2Th PID) -> Inner Loop/ Navigation/9(he2th PID)
  PID Gains [updated 4.28.16]/4(th2dE PID) -> Inner Loop/ Navigation/11(the2dE PID)
  PID Gains [updated 4.28.16]/5(Yaw Damp PID) -> Inner Loop/ Navigation/12(YawDamp PID)
  PID Gains [updated 4.28.16]/6(Roll PID) -> Inner Loop/ Navigation/13("Roll PID ")
  get Nav Vars [updated 4.28.16]/1("[phi the q r]") -> Demux1/1
  Demux1/1 -> Inner Loop/ Navigation/16(phi_m (rad))
  Demux1/2 -> Inner Loop/ Navigation/17(theta_m (rad))
  Inner Loop/ Navigation/7(theta_c) -> Terminator4/1
  Inner Loop/ Navigation/8(h_c_in) -> Terminator5/1
  Inner Loop/ Navigation/9(phi_c) -> Terminator6/1
  Demux1/4 -> Inner Loop/ Navigation/19(r_m (rad/s))
  Demux1/3 -> Inner Loop/ Navigation/18(q_m(rad))
  Trim Vals [updated 4.28.16]/5(Pil Console) -> [PilotCons]
  Inner Loop/ Navigation/1(dT(abs)) -> myMux Fun1/1(u1)
  Inner Loop/ Navigation/2(dA(rad)) -> myMux Fun1/2(u2)
  Inner Loop/ Navigation/3(dR(rad)) -> myMux Fun1/3(u3)
  Inner Loop/ Navigation/4(dE(rad)) -> myMux Fun1/4(u4)
  [PilotCons] -> Update PWM Commands and Send Telemetry [updated 4.27.16]/2(Pilot Console (IC) [dT dA dR dE])
  myMux Fun1/1(y) -> Update PWM Commands and Send Telemetry [updated 4.27.16]/1(PWM(rad) [dT dA dR dE])
  get Nav Vars [updated 4.28.16]/2(Euler Rot) -> [Euler_rot]
  get Nav Vars [updated 4.28.16]/3(PQR Rot) -> [PQR_rot]
  [Euler_rot] -> Update PWM Commands and Send Telemetry [updated 4.27.16]/3(Euler_rot)
  [PQR_rot] -> Update PWM Commands and Send Telemetry [updated 4.27.16]/4(PQR_rot)
  get Nav Vars [updated 4.28.16]/4(Yb Accel) -> Inner Loop/ Navigation/20(Yb Accel)
  [Pos_Hat] -> Inner Loop/ Navigation/21(XYZ (m))
  [Vned] -> Inner Loop/ Navigation/22(Vned (m/s))
  PID Gains [updated 4.28.16]/3(Roll2H FF) -> Inner Loop/ Navigation/10(Roll2H FF)
  PID Gains [updated 4.28.16]/7(dT FF) -> Inner Loop/ Navigation/14(dT FF gain)
  Trim Vals [updated 4.28.16]/6(Manual?) -> [isManual]
  [isManual] -> Inner Loop/ Navigation/23(Manual?)
  [isManual] -> Update PWM Commands and Send Telemetry [updated 4.27.16]/5(Manual?)
  Get RTB Order [navSupport.c] [updated 4.27.16]/1 -> Demux4/1
  Demux4/1 -> Inner Loop/ Navigation/33(RTB?)
  Demux4/2 -> Inner Loop/ Navigation/34(followMobile?)
  Trim Vals [updated 4.28.16]/7(V/I Sensor) -> [vISensor]
  [vISensor] -> Update PWM Commands and Send Telemetry [updated 4.27.16]/6(VI)
  [Accel] -> get Nav Vars [updated 4.28.16]/2(Accel)
  [Attitude] -> get Nav Vars [updated 4.28.16]/1(Attitude)
  [Accel_Bias] -> get Nav Vars [updated 4.28.16]/3(Accel. Bias)
  From20/1 -> Pilot LED and HIL Control Pins/2(HIL_Status)
  Inner Loop/ Navigation/6(ISR Loc) -> Terminator8/1
  Inner Loop/ Navigation/5("Puav ") -> Terminator7/1
  Get Max WP/1 -> Inner Loop/ Navigation/25(Max Wp Idx)
  Get mlMidLevelCommands/1 -> Inner Loop/ Navigation/1(U_c (m/s))
  Get mlMidLevelCommands/2 -> Inner Loop/ Navigation/2(h_c (m))
  Get mlMidLevelCommands/3 -> Inner Loop/ Navigation/3(psi_dot_c_man (rad))
  Get mlAirData/1 -> Inner Loop/ Navigation/15(dynP (Pa))
  isWpFly?/1 -> Inner Loop/ Navigation/24(wp Fly?)
  Mux/1 -> Inner Loop/ Navigation/35(Mobile Location)
  Get Mobile Location/2 -> Mux/2
  Get Mobile Location/1 -> Mux/1
  PAR_NAV_L2_BASE PAR_NAV_PRETURN_K PAR_NAV_SSCOMP_ON/2 -> Inner Loop/ Navigation/27(Turn LeadTime)
  PAR_NAV_L2_BASE PAR_NAV_PRETURN_K PAR_NAV_SSCOMP_ON/1 -> Inner Loop/ Navigation/26(T*  (m))
  PAR_NAV_L2_BASE PAR_NAV_PRETURN_K PAR_NAV_SSCOMP_ON/3 -> Inner Loop/ Navigation/28(SS Comp On)
  PAR_L1_OMEGA PAR_L1_M PAR_L1_GAMMA PAR_L1_ON_OFF/4 -> Inner Loop/ Navigation/32(L1OnOff)
  PAR_L1_OMEGA PAR_L1_M PAR_L1_GAMMA PAR_L1_ON_OFF/3 -> Inner Loop/ Navigation/31(gamma)
  PAR_L1_OMEGA PAR_L1_M PAR_L1_GAMMA PAR_L1_ON_OFF/2 -> Inner Loop/ Navigation/30(m)
  PAR_L1_OMEGA PAR_L1_M PAR_L1_GAMMA PAR_L1_ON_OFF/1 -> Inner Loop/ Navigation/29(omega)
  PAR_NAV_ISR_FAC PAR_PID_RMIX_ON PAR_PID_RMIX_P/1 -> Inner Loop/ Navigation/36(ISR Scale)
  PAR_NAV_ISR_FAC PAR_PID_RMIX_ON PAR_PID_RMIX_P/2 -> Inner Loop/ Navigation/37(dR Mix?)
  PAR_NAV_ISR_FAC PAR_PID_RMIX_ON PAR_PID_RMIX_P/3 -> Inner Loop/ Navigation/38(dR Mix Gain)
  isPassthrough/1 -> Passthrough Logic/1(In1)
  Passthrough Logic/1(Out1) -> Inner Loop/ Navigation/39(isPassthrough)
  Sensor_Data_Adapter/5(HIL On?) -> [HILON]
  Constant/1 -> HIL Manual Switch/1
  Constant1/1 -> HIL Manual Switch/2
  HIL Manual Switch/1 -> [HIL_FLAG]
  [HIL_FLAG] -> IMU_Mag_Driver/1(In1), Barometer_Driver/1(In1), Sensor_Data_Adapter/1(In1)
  [Position] -> To Control MCU/3(Position)
  [Biases] -> To Control MCU/4(Bias)
  [Attitude] -> To Control MCU/1(Attitude)
  [timeSt] -> To Control MCU/2(TimeSt)
  [Sensor] -> To Control MCU/5(SensorData)
  myMux Fun5/1(y) -> [Sensor]
  [Accel] -> myMux Fun5/1(u1)
  [Mag] -> myMux Fun5/2(u2)
  [Omega] -> myMux Fun5/3(u3)
  Get time4/1 -> [timeSt]
